simulink model "STEVE_Simulation_6DOF"  (R2025b)
settings: Solver=ode45  StartTime=0  StopTime=60  FixedStep=0.0001  MaxStep=0.0001  RelTol=1e-3
model workspace (MAT data in the model file):
  op_trim1 = opcond.OperatingReport
  op_trim1.TerminationString_ = 'Operating point specifications were successfully met.'
  op_trim1.OptimizationOutput_.iterations = 3
  op_trim1.OptimizationOutput_.funcCount = 171
  op_trim1.OptimizationOutput_.lssteplength = 1
  op_trim1.OptimizationOutput_.stepsize = 4.63262973918e-09
  op_trim1.OptimizationOutput_.algorithm = 'active-set'
  op_trim1.OptimizationOutput_.firstorderopt = 2.40097601741e-08
  op_trim1.OptimizationOutput_.constrviolation = 8.47716769092e-07
  op_trim1.OptimizationOutput_.message = 'Local minimum found that satisfies the constraints.
    | 
    | Optimization completed because the objective function is non-decreasing in 
    | feasible directions, to within the value of the optimality tolerance,
    | and constraints are satisfied to within the  value of the constraint tolerance.
    | 
    | <stopping criteria details>
    | 
    | Optimization completed: The first-order optimality measure, 2.400976e-08, is less
    | than options.OptimalityTolerance = 1.000000e-06, and the maximum constraint violation,
    | 8.477168e-07,is less than options.ConstraintTolerance = 1.000000e-06.'
  op_trim1.OptimizationOutput_.bestfeasible.x = [4290.04874097; 10725.1258376; 15852.6764872; 0.313155746169; -0.0981866680343; -0.0652604980678; 0.0059055243257; -0.636615168463; 8.14642489212e-06; -0.0176940249338; -0.00155509692213; -9.31199930506e-05; -0.000181100785288; 15.418172162; 0.559389025394; 3.31048087203; -37.2767340788; 1.38336022573; 8.21403291962e-06; 8.22046546553e-06; 8.22180678664e-06; 8.18637735168e-06; 8.165374813e-06; 8.15659926853e-06; 8.21875394544e-06; 8.19540646323e-06; 8.20244331077e-06; 8.1953609355e-06; 8.1983838895e-06; 8.22592390188e-06; 8.20694393928e-06; 8.20085018843e-06; 8.25311843786e-06; 8.2421945992e-06; 4.99999832196; 1.99999584909; 1.99999585143; 4.99999832977; 1.99999587773; 1.999995897; -0.000340053296214]
  op_trim1.OptimizationOutput_.bestfeasible.fval = 0
  op_trim1.OptimizationOutput_.bestfeasible.constrviolation = 8.47716769092e-07
  op_trim1.OptimizationOutput_.bestfeasible.firstorderopt = 2.40097601741e-08
  op_trim1.OptimizationOutput_.progress = {'<font face="monospaced"; size=3><BR>', 'Optimizing to solve for all desired dx/dt=0, x(k+1)-x(k)=0, and y=ydes.<BR>', ' <BR>', '(Maximum Error)  Block<BR>', ' ---------------------------------------------------------<BR>', '(3.86548e-01) STEVE_Simulation/STeVe System Model/Vehicle Dynamics/3DOF to 6DOF/Custom Variable Mass 3dof (Body Axes)<BR>', '(3.86551e-01) STEVE_Simulation/STeVe System Model/Vehicle Dynamics/3DOF to 6DOF/Custom Variable Mass 3dof (Body Axes)<BR>', '(8.47360e-07) STEVE_Simulation/STeVe System Model/Vehicle Dynamics/3DOF to 6DOF/Custom Variable Mass 3dof (Body Axes)<BR>', '(8.47764e-07) STEVE_Simulation/STeVe System Model/Vehicle Dynamics/3DOF to 6DOF/Custom Variable Mass 3dof (Body Axes)<BR>', '(8.47764e-07) STEVE_Simulation/STeVe System Model/Vehicle Dynamics/3DOF to 6DOF/Custom Variable Mass 3dof (Body Axes)<BR>', ' <BR>', 'Operating point specifications were successfully met.<BR>'}
  op_trim1.Model_ = 'STEVE_Simulation'
  op_trim1.States_(1) = opcond.StateReport
  op_trim1.States_(1).Nx_ = 1
  op_trim1.States_(1).Block_ = 'STEVE_Simulation/Environment/Wind/Discrete Wind Gust Model/Distance into
    | gust (x)/Distance into
    | Gust (x)
    | (Limited to gust length d)'
  op_trim1.States_(1).x_ = 1.999995897
  op_trim1.States_(1).SteadyState_ = 0
  op_trim1.States_(1).dxMin_ = -Inf
  op_trim1.States_(1).dxMax_ = Inf
  op_trim1.States_(1).Known_ = 0
  op_trim1.States_(1).Min_ = 0
  op_trim1.States_(1).Max_ = 2
  op_trim1.States_(2) = opcond.StateReport
  op_trim1.States_(2).Nx_ = 1
  op_trim1.States_(2).Block_ = 'STEVE_Simulation/Environment/Wind/Discrete Wind Gust Model/Distance into
    | gust (y)/Distance into
    | Gust (x)
    | (Limited to gust length d)
    | '
  op_trim1.States_(2).x_ = 1.99999587773
  op_trim1.States_(2).SteadyState_ = 0
  op_trim1.States_(2).dxMin_ = -Inf
  op_trim1.States_(2).dxMax_ = Inf
  op_trim1.States_(2).Known_ = 0
  op_trim1.States_(2).Min_ = 0
  op_trim1.States_(2).Max_ = 2
  op_trim1.States_(3) = opcond.StateReport
  op_trim1.States_(3).Nx_ = 1
  op_trim1.States_(3).Block_ = 'STEVE_Simulation/Environment/Wind/Discrete Wind Gust Model/Distance into
    | gust (z)/Distance into
    | Gust (x)
    | (Limited to gust length d)
    | '
  op_trim1.States_(3).x_ = 4.99999832977
  op_trim1.States_(3).SteadyState_ = 0
  op_trim1.States_(3).dxMin_ = -Inf
  op_trim1.States_(3).dxMax_ = Inf
  op_trim1.States_(3).Known_ = 0
  op_trim1.States_(3).Min_ = 0
  op_trim1.States_(3).Max_ = 5
  op_trim1.States_(4) = opcond.StateReport
  op_trim1.States_(4).Nx_ = 1
  op_trim1.States_(4).Block_ = 'STEVE_Simulation/Environment/Wind/Discrete Wind Gust Model1/Distance into
    | gust (x)/Distance into
    | Gust (x)
    | (Limited to gust length d)'
  op_trim1.States_(4).x_ = 1.99999585143
  op_trim1.States_(4).SteadyState_ = 0
  op_trim1.States_(4).dxMin_ = -Inf
  op_trim1.States_(4).dxMax_ = Inf
  op_trim1.States_(4).Known_ = 0
  op_trim1.States_(4).Min_ = 0
  op_trim1.States_(4).Max_ = 2
  op_trim1.States_(5) = opcond.StateReport
  op_trim1.States_(5).Nx_ = 1
  op_trim1.States_(5).Block_ = 'STEVE_Simulation/Environment/Wind/Discrete Wind Gust Model1/Distance into
    | gust (y)/Distance into
    | Gust (x)
    | (Limited to gust length d)
    | '
  op_trim1.States_(5).x_ = 1.99999584909
  op_trim1.States_(5).SteadyState_ = 0
  op_trim1.States_(5).dxMin_ = -Inf
  op_trim1.States_(5).dxMax_ = Inf
  op_trim1.States_(5).Known_ = 0
  op_trim1.States_(5).Min_ = 0
  op_trim1.States_(5).Max_ = 2
  op_trim1.States_(6) = opcond.StateReport
  op_trim1.States_(6).Nx_ = 1
  op_trim1.States_(6).Block_ = 'STEVE_Simulation/Environment/Wind/Discrete Wind Gust Model1/Distance into
    | gust (z)/Distance into
    | Gust (x)
    | (Limited to gust length d)
    | '
  op_trim1.States_(6).x_ = 4.99999832196
  op_trim1.States_(6).SteadyState_ = 0
  op_trim1.States_(6).dxMin_ = -Inf
  op_trim1.States_(6).dxMax_ = Inf
  op_trim1.States_(6).Known_ = 0
  op_trim1.States_(6).Min_ = 0
  op_trim1.States_(6).Max_ = 5
  op_trim1.States_(7) = opcond.StateReport
  op_trim1.States_(7).dx_ = [0; 0]
  op_trim1.States_(7).Nx_ = 2
  op_trim1.States_(7).Block_ = 'STEVE_Simulation/Environment/Wind/Dryden Wind Turbulence Model 
    | (Continuous (+q +r))/Filters on angular rates/Hpgw/pgw_p'
  op_trim1.States_(7).x_ = [8.25311843786e-06; 8.2421945992e-06]
  op_trim1.States_(7).SteadyState_ = [0; 0]
  op_trim1.States_(7).dxMin_ = [-Inf; -Inf]
  op_trim1.States_(7).dxMax_ = [Inf; Inf]
  op_trim1.States_(7).Known_ = [0; 0]
  op_trim1.States_(7).Min_ = [-Inf; -Inf]
  op_trim1.States_(7).Max_ = [Inf; Inf]
  op_trim1.States_(8) = opcond.StateReport
  op_trim1.States_(8).dx_ = [0; 0]
  op_trim1.States_(8).Nx_ = 2
  op_trim1.States_(8).Block_ = 'STEVE_Simulation/Environment/Wind/Dryden Wind Turbulence Model 
    | (Continuous (+q +r))/Filters on angular rates/Hqgw/qgw_p'
  op_trim1.States_(8).x_ = [8.20694393928e-06; 8.20085018843e-06]
  op_trim1.States_(8).SteadyState_ = [0; 0]
  op_trim1.States_(8).dxMin_ = [-Inf; -Inf]
  op_trim1.States_(8).dxMax_ = [Inf; Inf]
  op_trim1.States_(8).Known_ = [0; 0]
  op_trim1.States_(8).Min_ = [-Inf; -Inf]
  op_trim1.States_(8).Max_ = [Inf; Inf]
  op_trim1.States_(9) = opcond.StateReport
  op_trim1.States_(9).dx_ = [0; 0]
  op_trim1.States_(9).Nx_ = 2
  op_trim1.States_(9).Block_ = 'STEVE_Simulation/Environment/Wind/Dryden Wind Turbulence Model 
    | (Continuous (+q +r))/Filters on angular rates/Hrgw/rgw_p'
  op_trim1.States_(9).x_ = [8.1983838895e-06; 8.22592390188e-06]
  op_trim1.States_(9).SteadyState_ = [0; 0]
  op_trim1.States_(9).dxMin_ = [-Inf; -Inf]
  op_trim1.States_(9).dxMax_ = [Inf; Inf]
  op_trim1.States_(9).Known_ = [0; 0]
  op_trim1.States_(9).Min_ = [-Inf; -Inf]
  op_trim1.States_(9).Max_ = [Inf; Inf]
  op_trim1.States_(10) = opcond.StateReport
  op_trim1.States_(10).dx_ = [0; 0]
  op_trim1.States_(10).Nx_ = 2
  op_trim1.States_(10).Block_ = 'STEVE_Simulation/Environment/Wind/Dryden Wind Turbulence Model 
    | (Continuous (+q +r))/Filters on velocities/Hugw(s)/ug_p'
  op_trim1.States_(10).x_ = [8.20244331077e-06; 8.1953609355e-06]
  op_trim1.States_(10).SteadyState_ = [0; 0]
  op_trim1.States_(10).dxMin_ = [-Inf; -Inf]
  op_trim1.States_(10).dxMax_ = [Inf; Inf]
  op_trim1.States_(10).Known_ = [0; 0]
  op_trim1.States_(10).Min_ = [-Inf; -Inf]
  op_trim1.States_(10).Max_ = [Inf; Inf]
  op_trim1.States_(11) = opcond.StateReport
  op_trim1.States_(11).dx_ = [0; 0]
  op_trim1.States_(11).Nx_ = 2
  op_trim1.States_(11).Block_ = 'STEVE_Simulation/Environment/Wind/Dryden Wind Turbulence Model 
    | (Continuous (+q +r))/Filters on velocities/Hvgw(s)/vg_p1'
  op_trim1.States_(11).x_ = [8.165374813e-06; 8.15659926853e-06]
  op_trim1.States_(11).SteadyState_ = [0; 0]
  op_trim1.States_(11).dxMin_ = [-Inf; -Inf]
  op_trim1.States_(11).dxMax_ = [Inf; Inf]
  op_trim1.States_(11).Known_ = [0; 0]
  op_trim1.States_(11).Min_ = [-Inf; -Inf]
  op_trim1.States_(11).Max_ = [Inf; Inf]
  op_trim1.States_(12) = opcond.StateReport
  op_trim1.States_(12).dx_ = [0; 0]
  op_trim1.States_(12).Nx_ = 2
  op_trim1.States_(12).Block_ = 'STEVE_Simulation/Environment/Wind/Dryden Wind Turbulence Model 
    | (Continuous (+q +r))/Filters on velocities/Hvgw(s)/vgw_p2'
  op_trim1.States_(12).x_ = [8.21875394544e-06; 8.19540646323e-06]
  op_trim1.States_(12).SteadyState_ = [0; 0]
  op_trim1.States_(12).dxMin_ = [-Inf; -Inf]
  op_trim1.States_(12).dxMax_ = [Inf; Inf]
  op_trim1.States_(12).Known_ = [0; 0]
  op_trim1.States_(12).Min_ = [-Inf; -Inf]
  op_trim1.States_(12).Max_ = [Inf; Inf]
  op_trim1.States_(13) = opcond.StateReport
  op_trim1.States_(13).dx_ = [0; 0]
  op_trim1.States_(13).Nx_ = 2
  op_trim1.States_(13).Block_ = 'STEVE_Simulation/Environment/Wind/Dryden Wind Turbulence Model 
    | (Continuous (+q +r))/Filters on velocities/Hwgw(s)/wg_p1'
  op_trim1.States_(13).x_ = [8.21403291962e-06; 8.22046546553e-06]
  op_trim1.States_(13).SteadyState_ = [0; 0]
  op_trim1.States_(13).dxMin_ = [-Inf; -Inf]
  op_trim1.States_(13).dxMax_ = [Inf; Inf]
  op_trim1.States_(13).Known_ = [0; 0]
  op_trim1.States_(13).Min_ = [-Inf; -Inf]
  op_trim1.States_(13).Max_ = [Inf; Inf]
  op_trim1.States_(14) = opcond.StateReport
  op_trim1.States_(14).dx_ = [0; 0]
  op_trim1.States_(14).Nx_ = 2
  op_trim1.States_(14).Block_ = 'STEVE_Simulation/Environment/Wind/Dryden Wind Turbulence Model 
    | (Continuous (+q +r))/Filters on velocities/Hwgw(s)/wg_p2'
  op_trim1.States_(14).x_ = [8.22180678664e-06; 8.18637735168e-06]
  op_trim1.States_(14).SteadyState_ = [0; 0]
  op_trim1.States_(14).dxMin_ = [-Inf; -Inf]
  op_trim1.States_(14).dxMax_ = [Inf; Inf]
  op_trim1.States_(14).Known_ = [0; 0]
  op_trim1.States_(14).Min_ = [-Inf; -Inf]
  op_trim1.States_(14).Max_ = [Inf; Inf]
  op_trim1.States_(15) = opcond.StateReport
  op_trim1.States_(15).dx_ = [-1624.62107391; 4290.04874097; 10725.1258376]
  op_trim1.States_(15).Nx_ = 3
  op_trim1.States_(15).Block_ = 'STEVE_Simulation/GuidanceCommands/Transfer Fcn'
  op_trim1.States_(15).x_ = [4290.04874097; 10725.1258376; 15852.6764872]
  op_trim1.States_(15).SteadyState_ = [0; 0; 0]
  op_trim1.States_(15).dxMin_ = [-Inf; -Inf; -Inf]
  op_trim1.States_(15).dxMax_ = [Inf; Inf; Inf]
  op_trim1.States_(15).Known_ = [0; 0; 0]
  op_trim1.States_(15).Min_ = [-Inf; -Inf; -Inf]
  op_trim1.States_(15).Max_ = [Inf; Inf; Inf]
  op_trim1.States_(16) = opcond.StateReport
  op_trim1.States_(16).dx_ = -3.37116243602
  op_trim1.States_(16).Nx_ = 1
  op_trim1.States_(16).Block_ = 'STEVE_Simulation/STeVe System Model/Control System/Classical Upgraded/PID Controller1/Filter/Cont. Filter/Filter'
  op_trim1.States_(16).x_ = -0.00155509692213
  op_trim1.States_(16).SteadyState_ = 0
  op_trim1.States_(16).dxMin_ = -Inf
  op_trim1.States_(16).dxMax_ = Inf
  op_trim1.States_(16).Known_ = 0
  op_trim1.States_(16).Min_ = -Inf
  op_trim1.States_(16).Max_ = Inf
  op_trim1.States_(17) = opcond.StateReport
  op_trim1.States_(17).dx_ = -0.00991390700733
  op_trim1.States_(17).Nx_ = 1
  op_trim1.States_(17).Block_ = 'STEVE_Simulation/STeVe System Model/Control System/Classical Upgraded/PID Controller1/Integrator/Continuous/Integrator'
  op_trim1.States_(17).x_ = -0.0176940249338
  op_trim1.States_(17).SteadyState_ = 0
  op_trim1.States_(17).dxMin_ = -Inf
  op_trim1.States_(17).dxMax_ = Inf
  op_trim1.States_(17).Known_ = 0
  op_trim1.States_(17).Min_ = -Inf
  op_trim1.States_(17).Max_ = Inf
  op_trim1.States_(18) = opcond.StateReport
  op_trim1.States_(18).dx_ = 0.00151513100245
  op_trim1.States_(18).Nx_ = 1
  op_trim1.States_(18).Block_ = 'STEVE_Simulation/STeVe System Model/Control System/Classical Upgraded/PID Controller2/Filter/Cont. Filter/Filter'
  op_trim1.States_(18).x_ = 0.0059055243257
  op_trim1.States_(18).SteadyState_ = 0
  op_trim1.States_(18).dxMin_ = -Inf
  op_trim1.States_(18).dxMax_ = Inf
  op_trim1.States_(18).Known_ = 0
  op_trim1.States_(18).Min_ = -Inf
  op_trim1.States_(18).Max_ = Inf
  op_trim1.States_(19) = opcond.StateReport
  op_trim1.States_(19).dx_ = -0.037481221471
  op_trim1.States_(19).Nx_ = 1
  op_trim1.States_(19).Block_ = 'STEVE_Simulation/STeVe System Model/Control System/Classical Upgraded/PID Controller2/Integrator/Continuous/Integrator'
  op_trim1.States_(19).x_ = -0.0652604980678
  op_trim1.States_(19).SteadyState_ = 0
  op_trim1.States_(19).dxMin_ = -Inf
  op_trim1.States_(19).dxMax_ = Inf
  op_trim1.States_(19).Known_ = 0
  op_trim1.States_(19).Min_ = -Inf
  op_trim1.States_(19).Max_ = Inf
  op_trim1.States_(20) = opcond.StateReport
  op_trim1.States_(20).dx_ = -0.0747869203805
  op_trim1.States_(20).Nx_ = 1
  op_trim1.States_(20).Block_ = 'STEVE_Simulation/STeVe System Model/Control System/Classical Upgraded/PID Controller3/Filter/Cont. Filter/Filter'
  op_trim1.States_(20).x_ = -0.0981866680343
  op_trim1.States_(20).SteadyState_ = 0
  op_trim1.States_(20).dxMin_ = -Inf
  op_trim1.States_(20).dxMax_ = Inf
  op_trim1.States_(20).Known_ = 0
  op_trim1.States_(20).Min_ = -Inf
  op_trim1.States_(20).Max_ = Inf
  op_trim1.States_(21) = opcond.StateReport
  op_trim1.States_(21).dx_ = 0.273198142244
  op_trim1.States_(21).Nx_ = 1
  op_trim1.States_(21).Block_ = 'STEVE_Simulation/STeVe System Model/Control System/Classical Upgraded/PID Controller3/Integrator/Continuous/Integrator'
  op_trim1.States_(21).x_ = 0.313155746169
  op_trim1.States_(21).SteadyState_ = 0
  op_trim1.States_(21).dxMin_ = -Inf
  op_trim1.States_(21).dxMax_ = Inf
  op_trim1.States_(21).Known_ = 0
  op_trim1.States_(21).Min_ = -Inf
  op_trim1.States_(21).Max_ = Inf
  op_trim1.States_(22) = opcond.StateReport
  op_trim1.States_(22).dx_ = -0.000814642489212
  op_trim1.States_(22).Nx_ = 1
  op_trim1.States_(22).Block_ = 'STEVE_Simulation/STeVe System Model/Control System/Classical Upgraded/PID Controller6/Filter/Cont. Filter/Filter'
  op_trim1.States_(22).x_ = 8.14642489212e-06
  op_trim1.States_(22).SteadyState_ = 0
  op_trim1.States_(22).dxMin_ = -Inf
  op_trim1.States_(22).dxMax_ = Inf
  op_trim1.States_(22).Known_ = 0
  op_trim1.States_(22).Min_ = -Inf
  op_trim1.States_(22).Max_ = Inf
  op_trim1.States_(23) = opcond.StateReport
  op_trim1.States_(23).dx_ = -0.133481022202
  op_trim1.States_(23).Nx_ = 1
  op_trim1.States_(23).Block_ = 'STEVE_Simulation/STeVe System Model/Control System/Classical Upgraded/PID Controller6/Integrator/Continuous/Integrator'
  op_trim1.States_(23).x_ = -0.636615168463
  op_trim1.States_(23).SteadyState_ = 0
  op_trim1.States_(23).dxMin_ = -Inf
  op_trim1.States_(23).dxMax_ = Inf
  op_trim1.States_(23).Known_ = 0
  op_trim1.States_(23).Min_ = -Inf
  op_trim1.States_(23).Max_ = Inf
  op_trim1.States_(24) = opcond.StateReport
  op_trim1.States_(24).dx_ = 3.05199662227
  op_trim1.States_(24).Nx_ = 1
  op_trim1.States_(24).Block_ = 'STEVE_Simulation/STeVe System Model/Vehicle Dynamics/3DOF to 6DOF/Custom Variable Mass 3dof
    | (Body Axes)'
  op_trim1.States_(24).StateName_ = 'u'
  op_trim1.States_(24).x_ = 15.418172162
  op_trim1.States_(24).SteadyState_ = 0
  op_trim1.States_(24).dxMin_ = -Inf
  op_trim1.States_(24).dxMax_ = Inf
  op_trim1.States_(24).Known_ = 0
  op_trim1.States_(24).Min_ = -Inf
  op_trim1.States_(24).Max_ = Inf
  op_trim1.States_(25) = opcond.StateReport
  op_trim1.States_(25).dx_ = 1.82984252685
  op_trim1.States_(25).Nx_ = 1
  op_trim1.States_(25).Block_ = 'STEVE_Simulation/STeVe System Model/Vehicle Dynamics/3DOF to 6DOF/Custom Variable Mass 3dof
    | (Body Axes)'
  op_trim1.States_(25).StateName_ = 'w'
  op_trim1.States_(25).x_ = 0.559389025394
  op_trim1.States_(25).SteadyState_ = 0
  op_trim1.States_(25).dxMin_ = -Inf
  op_trim1.States_(25).dxMax_ = Inf
  op_trim1.States_(25).Known_ = 0
  op_trim1.States_(25).Min_ = -Inf
  op_trim1.States_(25).Max_ = Inf
  op_trim1.States_(26) = opcond.StateReport
  op_trim1.States_(26).dx_ = 3.42262162857
  op_trim1.States_(26).Nx_ = 1
  op_trim1.States_(26).Block_ = 'STEVE_Simulation/STeVe System Model/Vehicle Dynamics/3DOF to 6DOF/Custom Variable Mass 3dof
    | (Body Axes)'
  op_trim1.States_(26).StateName_ = 'Xe'
  op_trim1.States_(26).x_ = 3.31048087203
  op_trim1.States_(26).SteadyState_ = 0
  op_trim1.States_(26).dxMin_ = -Inf
  op_trim1.States_(26).dxMax_ = Inf
  op_trim1.States_(26).Known_ = 0
  op_trim1.States_(26).Min_ = -Inf
  op_trim1.States_(26).Max_ = Inf
  op_trim1.States_(27) = opcond.StateReport
  op_trim1.States_(27).dx_ = -15.0438894601
  op_trim1.States_(27).Nx_ = 1
  op_trim1.States_(27).Block_ = 'STEVE_Simulation/STeVe System Model/Vehicle Dynamics/3DOF to 6DOF/Custom Variable Mass 3dof
    | (Body Axes)'
  op_trim1.States_(27).StateName_ = 'Ze'
  op_trim1.States_(27).x_ = -37.2767340788
  op_trim1.States_(27).SteadyState_ = 0
  op_trim1.States_(27).dxMin_ = -Inf
  op_trim1.States_(27).dxMax_ = Inf
  op_trim1.States_(27).Known_ = 0
  op_trim1.States_(27).Min_ = -Inf
  op_trim1.States_(27).Max_ = Inf
  op_trim1.States_(28) = opcond.StateReport
  op_trim1.States_(28).dx_ = 8.47764429975e-07
  op_trim1.States_(28).Nx_ = 1
  op_trim1.States_(28).Block_ = 'STEVE_Simulation/STeVe System Model/Vehicle Dynamics/3DOF to 6DOF/Custom Variable Mass 3dof
    | (Body Axes)'
  op_trim1.States_(28).StateName_ = 'q'
  op_trim1.States_(28).SteadyState_ = 1
  op_trim1.States_(28).dxMin_ = -Inf
  op_trim1.States_(28).dxMax_ = Inf
  op_trim1.States_(28).Known_ = 1
  op_trim1.States_(28).Min_ = -Inf
  op_trim1.States_(28).Max_ = Inf
  op_trim1.States_(29) = opcond.StateReport
  op_trim1.States_(29).Nx_ = 1
  op_trim1.States_(29).Block_ = 'STEVE_Simulation/STeVe System Model/Vehicle Dynamics/3DOF to 6DOF/Custom Variable Mass 3dof
    | (Body Axes)'
  op_trim1.States_(29).StateName_ = 'theta'
  op_trim1.States_(29).x_ = 1.38336022573
  op_trim1.States_(29).SteadyState_ = 1
  op_trim1.States_(29).dxMin_ = -Inf
  op_trim1.States_(29).dxMax_ = Inf
  op_trim1.States_(29).Known_ = 0
  op_trim1.States_(29).Min_ = -Inf
  op_trim1.States_(29).Max_ = Inf
  op_trim1.States_(30) = opcond.StateReport
  op_trim1.States_(30).dx_ = -3.39724258746
  op_trim1.States_(30).Nx_ = 1
  op_trim1.States_(30).Block_ = 'STEVE_Simulation/STeVe System Model/Vehicle Dynamics/RocketEngineActuators/Delay'
  op_trim1.States_(30).x_ = -0.000340053296214
  op_trim1.States_(30).Ts_ = [0.0001 0]
  op_trim1.States_(30).SampleType_ = 'DSTATE'
  op_trim1.States_(30).SteadyState_ = 0
  op_trim1.States_(30).dxMin_ = -Inf
  op_trim1.States_(30).dxMax_ = Inf
  op_trim1.States_(30).Known_ = 0
  op_trim1.States_(30).Min_ = -Inf
  op_trim1.States_(30).Max_ = Inf
  op_trim1.States_(31) = opcond.StateReport
  op_trim1.States_(31).dx_ = [-0.000181100785288; -0.936056601197]
  op_trim1.States_(31).Nx_ = 2
  op_trim1.States_(31).Block_ = 'STEVE_Simulation/STeVe System Model/Vehicle Dynamics/RocketEngineActuators/Servo/Integrator,
    | Second-Order
    | Limited'
  op_trim1.States_(31).x_ = [-9.31199930506e-05; -0.000181100785288]
  op_trim1.States_(31).SteadyState_ = [0; 0]
  op_trim1.States_(31).dxMin_ = [-Inf; -Inf]
  op_trim1.States_(31).dxMax_ = [Inf; Inf]
  op_trim1.States_(31).Known_ = [0; 0]
  op_trim1.States_(31).Min_ = [-Inf; -Inf]
  op_trim1.States_(31).Max_ = [Inf; Inf]
undefined symbols (not defined in the file): Actuators, AeroData, C_inner_maxQ_d_Ki, C_inner_maxQ_d_Kp, C_outer_maxQ_d_Ki, C_outer_maxQ_d_Kp, F, launchpad_alt, Light, MIL, PrelookupData, Ref_Area, rocket_length, timeStep, Ts_inner, Ts_outer, warm_up_time, wn_ramp
libraries: simulink_extras x23, simulink x7, slpidlib x5, aerolibwind2 x3, aerolibconvert2 x3, aerolibasang x2, aerolibactuator x2, aerolibatmos2 x1
(part 1 of 2)
settings Model: SimulationMode=accelerator  ExtModeTrigDuration=2  Creator=jonno  LastModifiedBy=jonno
settings SolverCC: AutoInsertRateTranBlk=on
settings DataIOCC: ExternalInput=getinputstruct(op_trim1)  InitialState=getstatestruct(op_trim1)  SaveFormat=StructureWithTime
settings OptimizationCC: BlockReduction=off  BufferReuse=off
settings DebuggingCC: AlgebraicLoopMsg=none
settings HardwareCC: ProdBitPerLong=64.0  ProdHWDeviceType=Apple->ARM64
settings RTWCC: BuildConfiguration=Faster Runs
settings GRTTargetCC: RTWCAPISignals=on  RTWCAPIParams=on
settings ExplorerConfigSet: SimMechanicsOpenEditorOnUpdate=off

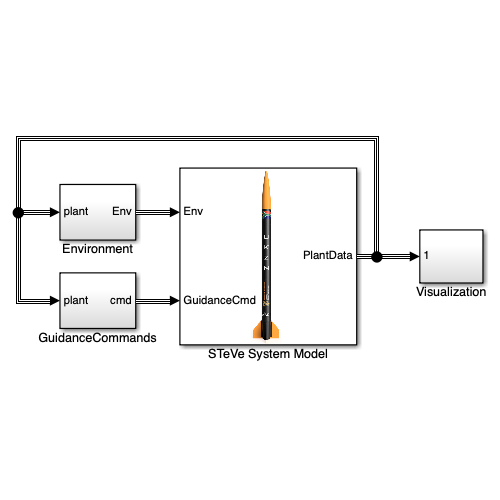
[thumbnail: Simulink's stored preview of the top-level diagram]
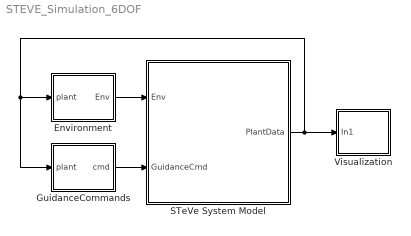
== system STEVE_Simulation_6DOF ==
  Environment : Subsystem
  GuidanceCommands : Subsystem
  STeVe System Model : Subsystem
      mask Display: image('/Users/jonno/MATLAB-Drive/masters-rocket-control-repository/simulation_6dof/docs/images/steve.png', [65 - (50 * (187 / 1041)), 0, 140 * (187 / 1041), 140])
  Visualization : Subsystem
  wires:
  GuidanceCommands/1(cmd) -> STeVe System Model/2(GuidanceCmd)
  Environment/1(Env) -> STeVe System Model/1(Env)
  STeVe System Model/1(PlantData) -> GuidanceCommands/1(plant), Environment/1(plant), Visualization/1(In1)

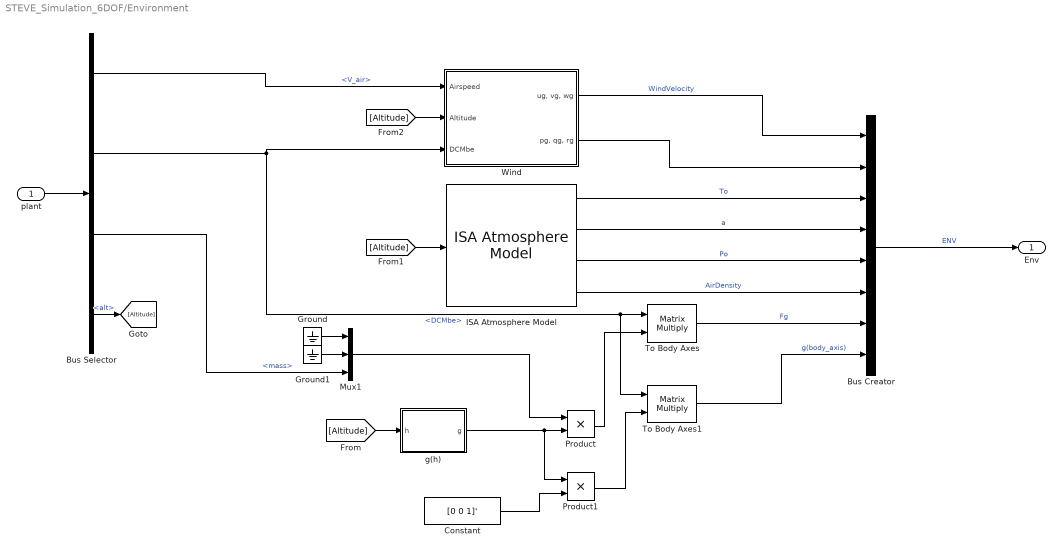
== system STEVE_Simulation_6DOF/Environment ==
  plant : Inport
  Bus Creator : BusCreator  Inputs=8
  Bus Selector : BusSelector  OutputSignals=V_air,DCMbe,mass,alt
  Constant : Constant  Value=[0 0 1]'
  Ground : Ground
  Ground1 : Ground
  ISA Atmosphere Model : aerolibatmos2/ISA Atmosphere Model  useExtended=on  action=None  custom=off  viscosityOut=off  g=9.80665  gamma=1.4  R=287.0531  L=0.0065  h_trop=11000  h_strat=20000  rho0=1.225  P0=101325  T0=288.15  h0=0  S=110.4  Tref=273.15  muref=1.716e-5
  Mux1 : Mux  Inputs=3
  Product : Product
  Product1 : Product
  To Body Axes : Product  Multiplication=Matrix(*)
  To Body Axes1 : Product  Multiplication=Matrix(*)
  Wind : Subsystem
  g(h) : MATLAB Function  TreatAsAtomicUnit=on
  Env : Outport
  wires:
  plant/1 -> Bus Selector/1
  Bus Creator/1 -> Env/1  "ENV"
  Bus Selector/3 -> Mux1/3  "<mass>"
  Ground/1 -> Mux1/1
  Ground1/1 -> Mux1/2
  Bus Selector/2 -> Wind/3(DCMbe), To Body Axes1/1, To Body Axes/1  "<DCMbe>"
  [Altitude] -> ISA Atmosphere Model/1
  To Body Axes/1 -> Bus Creator/7  "Fg"
  ISA Atmosphere Model/4 -> Bus Creator/6  "AirDensity"
  ISA Atmosphere Model/3 -> Bus Creator/5  "Po"
  ISA Atmosphere Model/2 -> Bus Creator/4  "a"
  ISA Atmosphere Model/1 -> Bus Creator/3  "To"
  [Altitude] -> Wind/2(Altitude)
  Wind/2("pg, qg, rg") -> Bus Creator/2
  Mux1/1 -> Product/1
  Product/1 -> To Body Axes/2
  [Altitude] -> g(h)/1(h)
  g(h)/1(g) -> Product1/1, Product/2
  Wind/1("ug, vg, wg") -> Bus Creator/1  "WindVelocity"
  Constant/1 -> Product1/2
  Product1/1 -> To Body Axes1/2
  To Body Axes1/1 -> Bus Creator/8  "g(body_axis)"
  Bus Selector/4 -> [Altitude]  "<alt>"
  Bus Selector/1 -> Wind/1(Airspeed)  "<V_air>"

== system STEVE_Simulation_6DOF/GuidanceCommands ==
  plant : Inport
  Bus Creator : BusCreator  Inputs=4
  Constant : Constant  Value=90
  Constant1 : Constant  Value=0
  Degrees to Radians : simulink_extras/Transformations/Degrees to Radians
  Degrees to Radians1 : simulink_extras/Transformations/Degrees to Radians
  Rate Limiter : RateLimiter  RisingSlewLimit=2000/60  FallingSlewLimit=-0.5  SampleTimeMode=inherited
  Rate Limiter2 : RateLimiter  RisingSlewLimit=0.5  FallingSlewLimit=-0.5  SampleTimeMode=inherited
  Step : Step  After=2000  SampleTime=0
  ThrottleCmd % : Step  Time=Actuators.Engine.BurnTime  Before=1  After=0.0001  SampleTime=0  VectorParams1D=off
  cmd : Outport
  wires:
  Bus Creator/1 -> cmd/1  "CMD"
  Degrees to Radians/1 -> Bus Creator/2  "theta_cmd"
  ThrottleCmd %/1 -> Rate Limiter2/1  "ThrottleCmd"
  Rate Limiter2/1 -> Bus Creator/1  "throttle_cmd"
  Constant/1 -> Degrees to Radians/1
  Step/1 -> Rate Limiter/1
  Rate Limiter/1 -> Bus Creator/4  "Xe_Cmd"
  Constant1/1 -> Degrees to Radians1/1
  Degrees to Radians1/1 -> Bus Creator/3  "psi_cmd"

== system STEVE_Simulation_6DOF/STeVe System Model ==
  Env : Inport
  GuidanceCmd : Inport  Port=2
  Env1 : InportShadow
  State Estimator : Subsystem
  Subsystem : Subsystem
  Vehicle Dynamics : Subsystem
  PlantData : Outport
  wires:
  Env/1 -> Vehicle Dynamics/1(Env)
  Vehicle Dynamics/1(PlantData) -> Subsystem/3(PlantData), State Estimator/2(Plant), PlantData/1  "Plant"
  GuidanceCmd/1 -> Subsystem/1(GuidanceCommandBus)
  Env1/1 -> State Estimator/1(Env)
  State Estimator/1(Sensors) -> Subsystem/2(Sensors)
  Subsystem/1(ActCmd) -> Vehicle Dynamics/2(ActCmd)

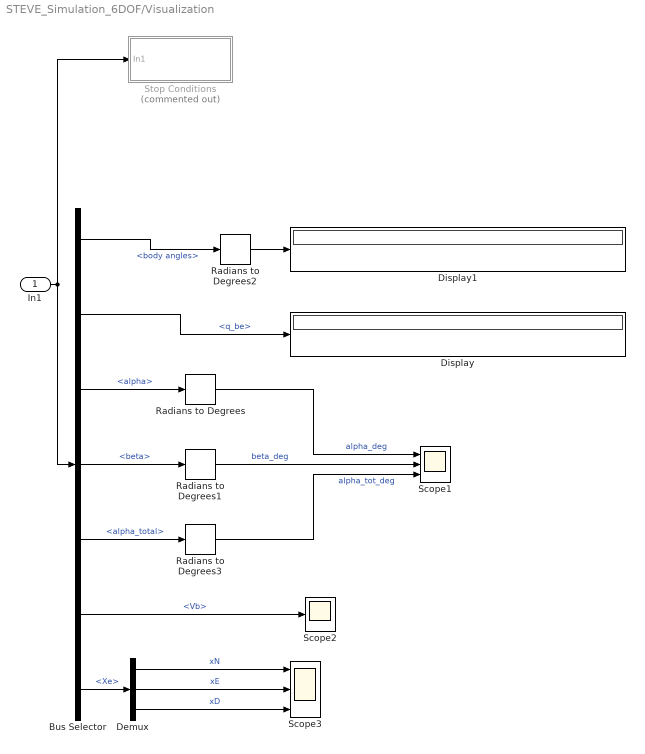
== system STEVE_Simulation_6DOF/Visualization ==
  In1 : Inport
  Bus Selector : BusSelector  OutputSignals=body angles,q_be,alpha,beta,alpha_total,Vb,Xe
  Demux : Demux  Outputs=3
  Display : Display
  Display1 : Display
  Radians to Degrees{,1..3} (4 alike) : simulink_extras/Transformations/Radians to Degrees
  Scope1 : Scope  NumInputPorts=3
      settings: ActiveDisplayYMinimum=0.52794946772114626  ActiveDisplayYMaximum=0.85095852928901983  DataLoggingVariableName=ScopeData3
  Scope2 : Scope
      settings: ActiveDisplayYMinimum=-0.64239324283240506  ActiveDisplayYMaximum=0.59138262660134089  DataLoggingVariableName=ScopeData4
  Scope3 : Scope  NumInputPorts=3
      settings: ActiveDisplayYMinimum=-1.7095998760294862  ActiveDisplayYMaximum=2.8596467575037732
  Stop Conditions : Subsystem  Commented=on
  wires:
  In1/1 -> Stop Conditions/1(In1), Bus Selector/1
  Bus Selector/1 -> Radians to Degrees2/1  "<body angles>"
  Bus Selector/3 -> Radians to Degrees/1  "<alpha>"
  Bus Selector/4 -> Radians to Degrees1/1  "<beta>"
  Radians to Degrees/1 -> Scope1/1  "alpha_deg"
  Radians to Degrees1/1 -> Scope1/2  "beta_deg"
  Bus Selector/6 -> Scope2/1  "<Vb>"
  Bus Selector/2 -> Display/1  "<q_be>"
  Radians to Degrees2/1 -> Display1/1
  Bus Selector/7 -> Demux/1  "<Xe>"
  Demux/2 -> Scope3/2  "xE"
  Demux/1 -> Scope3/1  "xN"
  Demux/3 -> Scope3/3  "xD"
  Bus Selector/5 -> Radians to Degrees3/1  "<alpha_total>"
  Radians to Degrees3/1 -> Scope1/3  "alpha_tot_deg"

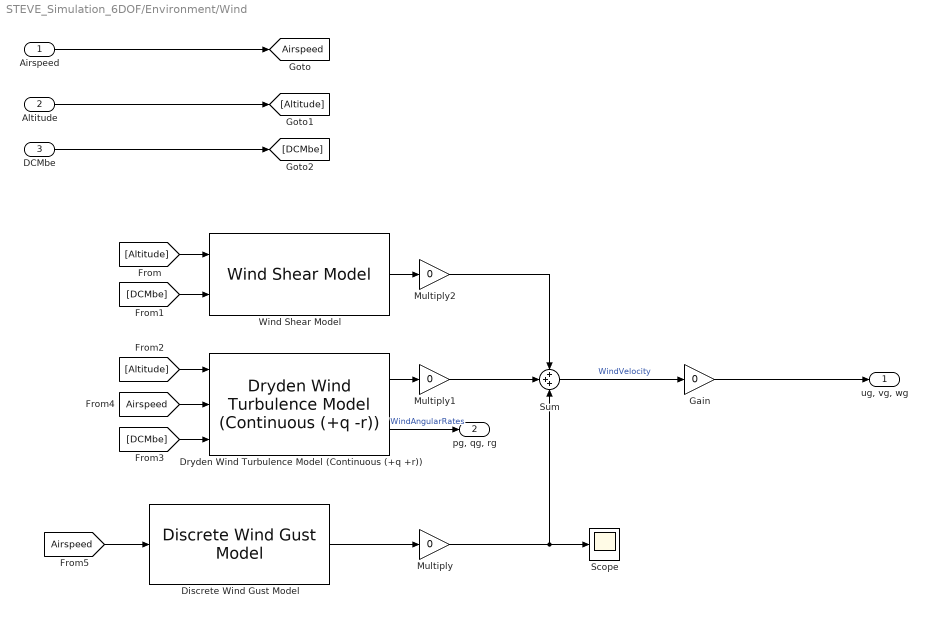
== system STEVE_Simulation_6DOF/Environment/Wind ==
  Airspeed : Inport
  Altitude : Inport  Port=2
  DCMbe : Inport  Port=3
  Discrete Wind Gust Model : aerolibwind2/Discrete Wind Gust Model  units=Metric (MKS)  Gx=on  Gy=off  Gz=off  t_0=1  d_m=[50 10 10]  v_m=[30 0 0]
  Dryden Wind Turbulence Model (Continuous (+q +r)) : aerolibwind2/Dryden Wind Turbulence Model  (Continuous (+q -r))  units=Metric (MKS)  spec=MIL-F-8785C  model=Continuous Dryden (+q +r)  W20=15  Wdeg=0  TurbProb=10^-2 - Light  L_high=533.4  Wingspan=10  ts=0.1  Seed=[23341 23342 23343 23344]  T_on=off
      settings: LibrarySourceBlock=|
      | aerolibwind2/Dryden Wind Turbulence Model
      | (Continuous (+q +r))
  Gain : Gain  Gain=0
  Multiply : Gain  Gain=0
  Multiply1 : Gain  Gain=0
  Multiply2 : Gain  Gain=0
  Scope : Scope
      settings: ActiveDisplayYMinimum=-3.4473346269998206  ActiveDisplayYMaximum=16.02681366587808  DataLoggingVariableName=ScopeData5
  Sum : Sum  Inputs=+++
  Wind Shear Model : aerolibwind2/Wind Shear Model  units=Metric (MKS)  phase=Category C - Terminal Flight Phase  W_20=Wind.shear  Wdeg=90
  "ug, vg, wg" : Outport
  "pg, qg, rg" : Outport  Port=2
  tag scope: Airspeed=global
  wires:
  DCMbe/1 -> [DCMbe]
  [Altitude] -> Wind Shear Model/1
  [DCMbe] -> Wind Shear Model/2
  [Altitude] -> Dryden Wind Turbulence Model (Continuous (+q +r))/1
  [DCMbe] -> Dryden Wind Turbulence Model (Continuous (+q +r))/3
  [Airspeed] -> Dryden Wind Turbulence Model (Continuous (+q +r))/2
  [Airspeed] -> Discrete Wind Gust Model/1
  Sum/1 -> Gain/1  "WindVelocity"
  Dryden Wind Turbulence Model (Continuous (+q +r))/2 -> "pg, qg, rg"/1  "WindAngularRates"
  Altitude/1 -> [Altitude]
  Multiply/1 -> Sum/3, Scope/1
  Wind Shear Model/1 -> Multiply2/1
  Dryden Wind Turbulence Model (Continuous (+q +r))/1 -> Multiply1/1
  Multiply1/1 -> Sum/2
  Multiply2/1 -> Sum/1
  Discrete Wind Gust Model/1 -> Multiply/1
  Airspeed/1 -> [Airspeed]
  Gain/1 -> "ug, vg, wg"/1

== system STEVE_Simulation_6DOF/STeVe System Model/State Estimator ==
  note: We need to estimate Qbar
  Env : Inport
  Plant : Inport  Port=2
  Bus Creator : BusCreator  Inputs=3
  Bus Selector : BusSelector  OutputSignals=lat,long,alt,Ve,Ab,w,DCMbe,body angles,V_air
  Bus Selector1 : BusSelector  OutputSignals=g(body_axis),AirDensity
  Sensors : Outport
  wires:
  Plant/1 -> Bus Selector/1
  Env/1 -> Bus Selector1/1
  Bus Creator/1 -> Sensors/1
  [qbar] -> Bus Creator/3

== system STEVE_Simulation_6DOF/STeVe System Model/Subsystem ==
  GuidanceCommandBus : Inport
  Sensors : Inport  Port=2
  PlantData : Inport  Port=3
  Classical Upgraded : Subsystem
  Classical Upgraded1 : Subsystem  Commented=on
  ActCmd : Outport
  wires:
  Sensors/1 -> Classical Upgraded/2(Sensors)
  PlantData/1 -> Classical Upgraded/1(PlantData)
  Classical Upgraded/1(Cmd Out) -> ActCmd/1
  GuidanceCommandBus/1 -> Classical Upgraded/3(CMD)

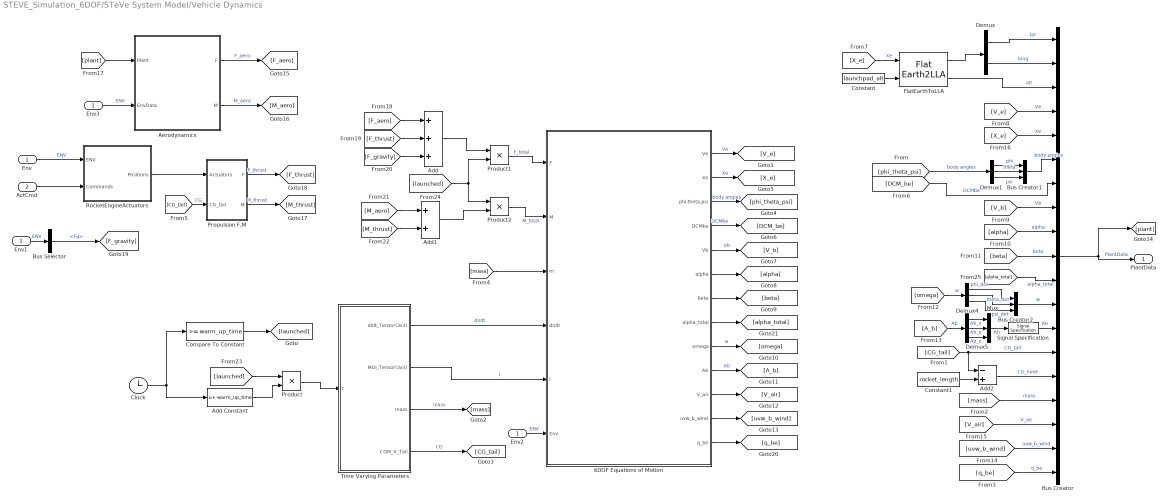
== system STEVE_Simulation_6DOF/STeVe System Model/Vehicle Dynamics ==
  Env : Inport
  ActCmd : Inport  Port=2
  6DOF Equations of Motion : Subsystem
  Add : Sum  Inputs=+++
  Add Constant : Bias  Bias=-warm_up_time  SaturateOnIntegerOverflow=off
  Add1 : Sum
  Add2 : Sum  Inputs=-+
  Aerodynamics : Subsystem
  Bus Creator : BusCreator  Inputs=19
  Bus Creator1 : BusCreator  Inputs=3
  Bus Creator2 : BusCreator  Inputs=3
  Bus Selector : BusSelector  OutputSignals=Fg
  Clock : Clock
  Compare To Constant : simulink/Logic and Bit Operations/Compare To Constant  relop=>=  const=warm_up_time  OutDataTypeStr=boolean
  Constant : Constant  Value=launchpad_alt
  Constant1 : Constant  Value=rocket_length
  Demux : Demux  Outputs=2
  Demux1 : Demux  Outputs=3
  Demux4 : Demux  Outputs=3
  Demux5 : Demux  Outputs=3
  Env1 : InportShadow
  Env2 : InportShadow
  Env3 : InportShadow
  FlatEarthToLLA : FlatEarth2LLA  R=6378137
  Mux : Mux  Inputs=3
  Product : Product
  Product1 : Product
  Product2 : Product
  Propulsion F,M : Subsystem
  RocketEngineActuators : Subsystem
  Signal Specification : SignalSpecification  Dimensions=[1 3]
  Time Varying Parameters : Subsystem
  PlantData : Outport
  wires:
  ActCmd/1 -> RocketEngineActuators/2(Commands)
  RocketEngineActuators/1(Positions) -> Propulsion F,M/1(Actuators)
  Bus Creator/1 -> [plant], PlantData/1  "PlantData"
  [X_e] -> FlatEarthToLLA/1  "Xe"
  Demux/1 -> Bus Creator/1  "lat"
  Demux/2 -> Bus Creator/2  "long"
  FlatEarthToLLA/1 -> Demux/1
  FlatEarthToLLA/2 -> Bus Creator/3  "alt"
  [V_e] -> Bus Creator/4  "Ve"
  [phi_theta_psi] -> Demux1/1  "body angles"
  Demux1/1 -> Bus Creator1/1  "phi"
  Demux1/2 -> Bus Creator1/2  "theta"
  Demux1/3 -> Bus Creator1/3  "psi"
  Bus Creator1/1 -> Bus Creator/6  "body angles"
  [DCM_be] -> Bus Creator/7  "DCMbe"
  [V_b] -> Bus Creator/8  "Vb"
  [alpha] -> Bus Creator/9  "alpha"
  [beta] -> Bus Creator/10  "beta"
  [omega] -> Demux4/1  "w"
  Signal Specification/1 -> Bus Creator/13  "Ab"
  Propulsion F,M/1(F) -> [F_thrust]  "F_thrust"
  [CG_tail] -> Bus Creator/14, Add2/1  "CG_tail"
  [mass] -> Bus Creator/16  "mass"
  Env/1 -> RocketEngineActuators/1(ENV)  "ENV"
  Propulsion F,M/2(M) -> [M_thrust]  "M_thrust"
  Clock/1 -> Add Constant/1, Compare To Constant/1
  Time Varying Parameters/1(dIdt_Tensor(3x3)) -> 6DOF Equations of Motion/4(dI/dt)  "dI/dt"
  Time Varying Parameters/2(MOI_Tensor(3x3)) -> 6DOF Equations of Motion/5(I)  "I"
  Time Varying Parameters/3(mass) -> [mass]  "mass"
  Time Varying Parameters/4(COM_X_Tail) -> [CG_tail]  "CG"
  [mass] -> 6DOF Equations of Motion/3(m)
  Product1/1 -> 6DOF Equations of Motion/1(F)  "F_total"
  Aerodynamics/1(F) -> [F_aero]  "F_aero"
  Env2/1 -> 6DOF Equations of Motion/6(Env)  "ENV"
  [CG_tail] -> Propulsion F,M/2(CG_tail)  "CG"
  Aerodynamics/2(M) -> [M_aero]  "M_aero"
  [uvw_b_wind] -> Bus Creator/18  "uvw_b_wind"
  Demux4/1 -> Bus Creator2/1  "phi_dot"
  Demux4/3 -> Bus Creator2/3  "psi_dot"
  Demux4/2 -> Bus Creator2/2  "theta_dot"
  Bus Creator2/1 -> Bus Creator/12  "w"
  Demux5/1 -> Mux/1  "Ab_x"
  Demux5/2 -> Mux/2  "Ab_y"
  Demux5/3 -> Mux/3  "Ab_z"
  [A_b] -> Demux5/1  "Ab"
  Mux/1 -> Signal Specification/1  "Ab"
  Product2/1 -> 6DOF Equations of Motion/2(M)  "M_total"
  Constant/1 -> FlatEarthToLLA/2
  6DOF Equations of Motion/1(Ve) -> [V_e]  "Ve"
  6DOF Equations of Motion/3(phi,theta,psi) -> [phi_theta_psi]  "body angles"
  6DOF Equations of Motion/2(Xe) -> [X_e]  "Xe"
  6DOF Equations of Motion/4(DCMbe) -> [DCM_be]  "DCMbe"
  6DOF Equations of Motion/5(Vb) -> [V_b]  "Vb"
  6DOF Equations of Motion/6(alpha) -> [alpha]
  6DOF Equations of Motion/7(beta) -> [beta]
  6DOF Equations of Motion/9(omega) -> [omega]  "w"
  6DOF Equations of Motion/10(Ab) -> [A_b]  "Ab"
  6DOF Equations of Motion/11(V_air) -> [V_air]
  6DOF Equations of Motion/12(uvw_b_wind) -> [uvw_b_wind]
  [V_air] -> Bus Creator/17  "V_air"
  [X_e] -> Bus Creator/5  "Xe"
  [plant] -> Aerodynamics/1(Plant)
  Env3/1 -> Aerodynamics/2(EnvData)  "ENV"
  Env1/1 -> Bus Selector/1  "ENV"
  Bus Selector/1 -> [F_gravity]  "<Fg>"
  [F_aero] -> Add/1
  [F_thrust] -> Add/2
  [F_gravity] -> Add/3
  [M_aero] -> Add1/1
  [M_thrust] -> Add1/2
  Compare To Constant/1 -> [launched]
  [launched] -> Product/1
  Product/1 -> Time Varying Parameters/1(t)
  Add/1 -> Product1/1
  Add1/1 -> Product2/2
  [launched] -> Product2/1, Product1/2
  Add Constant/1 -> Product/2
  Constant1/1 -> Add2/2
  Add2/1 -> Bus Creator/15  "CG_nose"
  6DOF Equations of Motion/13(q_be) -> [q_be]
  [q_be] -> Bus Creator/19  "q_be"
  6DOF Equations of Motion/8(alpha_total) -> [alpha_total]
  [alpha_total] -> Bus Creator/11  "alpha_total"

== system STEVE_Simulation_6DOF/Visualization/Stop Conditions ==
  In1 : Inport
  AND : Logic  IconShape=distinctive  AllPortsSameDT=off  OutDataTypeStr=boolean
  Abs : Abs  SaturateOnIntegerOverflow=off
  Abs1 : Abs  SaturateOnIntegerOverflow=off
  Bus Selector : BusSelector  OutputSignals=alpha,beta
  Clock : Clock
  Compare To Constant : simulink/Logic and Bit Operations/Compare To Constant  relop=>=  const=40  OutDataTypeStr=boolean
  Compare To Constant1 : simulink/Logic and Bit Operations/Compare To Constant  relop=>=  const=warm_up_time  OutDataTypeStr=boolean
  Max : MinMax  Function=max  Inputs=2
  Radians to Degrees : simulink_extras/Transformations/Radians to Degrees
  Stop Simulation : Stop
  wires:
  In1/1 -> Bus Selector/1
  Bus Selector/1 -> Abs/1  "<alpha>"
  Bus Selector/2 -> Abs1/1  "<beta>"
  Max/1 -> Radians to Degrees/1
  Radians to Degrees/1 -> Compare To Constant/1
  Compare To Constant/1 -> AND/2
  Abs/1 -> Max/1
  Abs1/1 -> Max/2
  AND/1 -> Stop Simulation/1
  Clock/1 -> Compare To Constant1/1
  Compare To Constant1/1 -> AND/1

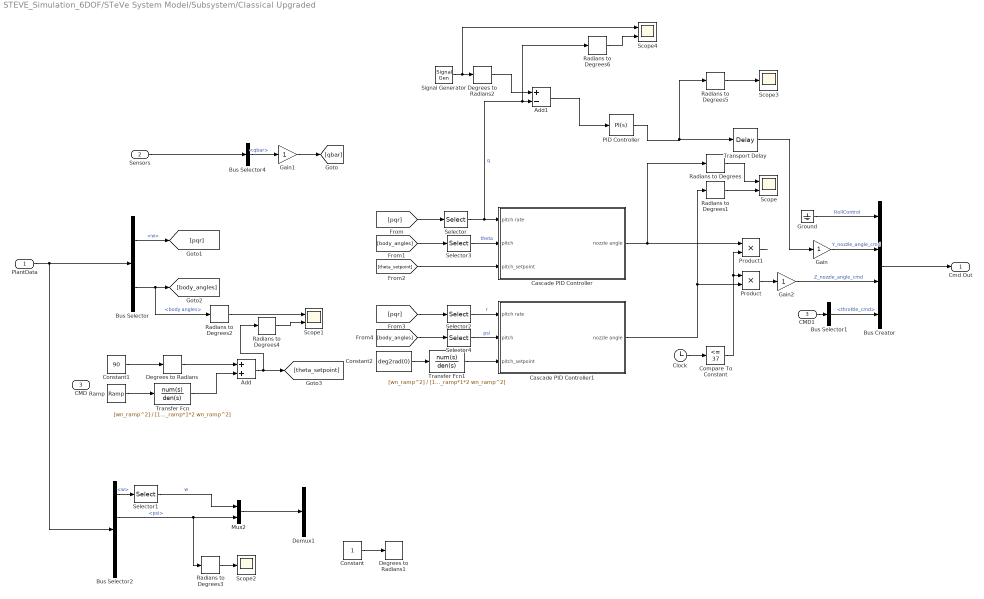
== system STEVE_Simulation_6DOF/STeVe System Model/Subsystem/Classical Upgraded ==
  PlantData : Inport
  Sensors : Inport  Port=2
  CMD : Inport  Port=3
  Add : Sum
  Add1 : Sum  Inputs=+-
  Bus Creator : BusCreator  Inputs=4
  Bus Selector : BusSelector  OutputSignals=w,body angles
  Bus Selector1 : BusSelector  OutputSignals=throttle_cmd
  Bus Selector2 : BusSelector  OutputSignals=w,body angles.psi,Ve,V_air
  Bus Selector4 : BusSelector  OutputSignals=qbar
  CMD1 : InportShadow  Port=3
  Cascade PID Controller : Subsystem
  Cascade PID Controller1 : Subsystem
  Clock : Clock
  Compare To Constant : simulink/Logic and Bit Operations/Compare To Constant  relop=<=  const=37  OutDataTypeStr=boolean
  Constant : Constant
  Constant1 : Constant  Value=90
  Constant2 : Constant  Value=deg2rad(0)
  Degrees to Radians : simulink_extras/Transformations/Degrees to Radians
  Degrees to Radians1 : simulink_extras/Transformations/Degrees to Radians
  Degrees to Radians2 : simulink_extras/Transformations/Degrees to Radians
  Demux1 : Demux  Outputs=2
  Gain : Gain
  Gain1 : Gain
  Gain2 : Gain
  Ground : Ground
  Mux2 : Mux  Inputs=2
  PID Controller : slpidlib/PID Controller  Controller=PI  Form=Parallel  TimeDomain=Continuous-time  UseExternalTs=off  SampleTime=-1  IntegratorMethod=Forward Euler  FilterMethod=Forward Euler  ControllerParametersSource=internal  P=1.8265  I=14.0169  UseKiTs=off  D=0  UseExternalDerivativeSource=off  N=100  UseFilter=on  TunerSelectOption=Transfer Function Based (PID Tuner App)  InitialConditionSource=internal  InitialConditionForIntegrator=0  InitialConditionForFilter=0  DifferentiatorICPrevScaledInput=0  ExternalReset=none  TrackingMode=off  Kt=1  LimitOutput=off  SatLimitsSource=internal  UpperSaturationLimit=inf  LowerSaturationLimit=-inf  LinearizeAsGain=on  AntiWindupMode=none  Kb=1  LimitIntegrator=off  UpperIntegratorSaturationLimit=inf  LowerIntegratorSaturationLimit=-inf  POutMin=[]  POutMax=[]  IOutMin=[]  IOutMax=[]  DOutMin=[]  DOutMax=[]  NOutMin=[]  NOutMax=[]  SumOutMin=[]  SumOutMax=[]  SaturationOutMin=[]  SaturationOutMax=[]  PParamMin=[]  PParamMax=[]  IParamMin=[]  IParamMax=[]  DParamMin=[]  DParamMax=[]  NParamMin=[]  NParamMax=[]  KbParamMin=[]  KbParamMax=[]  KtParamMin=[]  KtParamMax=[]  KbOutMin=[]  KbOutMax=[]  KtOutMin=[]  KtOutMax=[]  IntegratorOutMin=[]  IntegratorOutMax=[]  FilterOutMin=[]  FilterOutMax=[]  SumI1OutMin=[]  SumI1OutMax=[]  SumI2OutMin=[]  SumI2OutMax=[]  SumI3OutMin=[]  SumI3OutMax=[]  SumI4OutMin=[]  SumI4OutMax=[]  SumDOutMin=[]  SumDOutMax=[]  DifferentiatorOutMin=[]  DifferentiatorOutMax=[]  FilterDiffOutCoefMin=[]  FilterDiffOutCoefMax=[]  ReciprocalOutMin=[]  ReciprocalOutMax=[]  SumDenOutMin=[]  SumDenOutMax=[]  SumNumOutMin=[]  SumNumOutMax=[]  DivideOutMin=[]  DivideOutMax=[]  UdiffTsProdOutMin=[]  UdiffTsProdOutMax=[]  NTsProdOutMin=[]  NTsProdOutMax=[]  UintegralTsProdOutMin=[]  UintegralTsProdOutMax=[]  UngainTsProdOutMin=[]  UngainTsProdOutMax=[]  ClampingZeroOutDataTypeStr=Inherit: Inherit via back propagation  ClampingZeroOutMin=[]  ClampingZeroOutMax=[]  FilterDenConstantOutDataTypeStr=Inherit: Inherit via back propagation  FilterDenConstantOutMin=[]  FilterDenConstantOutMax=[]  PCopyOutDataTypeStr=Inherit: Inherit via back propagation  PCopyOutMin=[]  PCopyOutMax=[]  NCopyOutDataTypeStr=Inherit: Inherit via back propagation  NCopyOutMin=[]  NCopyOutMax=[]  IntegratorContinuousStateAttributes=''  IntegratorStateMustResolveToSignalObject=off  IntegratorRTWStateStorageClass=Auto  FilterContinuousStateAttributes=''  FilterStateMustResolveToSignalObject=off  FilterRTWStateStorageClass=Auto  ParallelPVariant=InternalParameters  IdealPVariant=Disabled  IVariant=InternalParameters  DVariant=Disabled  IntegratorVariant=Continuous  SatVariant=Disabled  AWVariant=Passthrough  PCopyVariant=Disabled  TRVariant=Disabled  FdbkBlocksVariant=Forward  IdealPFdbkVariant=Disabled  SatFdbkVariant=Disabled  DerivativeFilterVariant=Disabled  NVariant=Disabled  NCopyVariant=Disabled_SignalSpec  FilterICVariant=Disabled  IntegratorICVariant=InternalICs  ExternalResetVariant=Disabled  TRSumVariant=Passthrough  SumFdbkVariant=Disabled  SumVariant=Sum_PI  TsampFilterVariant=InternalTs  TsampNgainVariant=Passthrough  TsampIntegralVariant=Disabled_SignalSpec  ExternalSaturationOutDataTypeStr=Inherit: Same as second input  DerivativeSourceVariant=Disabled  PreIntVariant=InternalPreInt
  Product : Product
  Product1 : Product
  Radians to Degrees{,1..6} (7 alike) : simulink_extras/Transformations/Radians to Degrees
  Ramp : simulink/Sources/Ramp  slope=-(10/60)*pi/180  start=0  InitialOutput=0
  Scope : Scope  NumInputPorts=2
      settings: ActiveDisplayYMinimum=-2.0223368539006419  ActiveDisplayYMaximum=0.30837107460030577  DataLoggingVariableName=ScopeData10
  Scope1 : Scope  NumInputPorts=2
      settings: ActiveDisplayYMinimum=-85.342848172773913  ActiveDisplayYMaximum=210.22972215938358  DataLoggingVariableName=ScopeData11
  Scope2 : Scope
      settings: ActiveDisplayYMinimum=-18.362797933212903  ActiveDisplayYMaximum=16.52585265642092  DataLoggingVariableName=ScopeData7
  Scope3 : Scope
      settings: ActiveDisplayYMinimum=-2535.4711139327528  ActiveDisplayYMaximum=531.06890360245575  DataLoggingVariableName=ScopeData12
  Scope4 : Scope  NumInputPorts=2
      settings: ActiveDisplayYMinimum=-83.658192950020577  ActiveDisplayYMaximum=117.69725689081616  DataLoggingVariableName=ScopeData13
  Selector : Selector  InputPortWidth=3  IndexOptions=Index vector (dialog)  Indices=[2]  OutputSizes=1
  Selector1 : Selector  InputPortWidth=3  IndexOptions=Index vector (dialog)  Indices=[3]  OutputSizes=1
  Selector2 : Selector  InputPortWidth=3  IndexOptions=Index vector (dialog)  Indices=[3]  OutputSizes=1
  Selector3 : Selector  InputPortWidth=3  IndexOptions=Index vector (dialog)  Indices=[2]  OutputSizes=1
  Selector4 : Selector  InputPortWidth=3  IndexOptions=Index vector (dialog)  Indices=[3]  OutputSizes=1
  Signal Generator : SignalGenerator  Amplitude=10  Frequency=0.5
  Transfer Fcn : TransferFcn  Numerator=[wn_ramp^2]  Denominator=[1 wn_ramp*1*2 wn_ramp^2]
  Transfer Fcn1 : TransferFcn  Numerator=[wn_ramp^2]  Denominator=[1 wn_ramp*1*2 wn_ramp^2]
  Transport Delay : TransportDelay  DelayTime=0.05
  Cmd Out : Outport
  wires:
  Gain/1 -> Bus Creator/2  "Y_nozzle_angle_cmd"
  Ground/1 -> Bus Creator/1  "RollControl"
  Bus Creator/1 -> Cmd Out/1
  CMD1/1 -> Bus Selector1/1
  Bus Selector1/1 -> Bus Creator/4  "<throttle_cmd>"
  Ramp/1 -> Transfer Fcn/1
  Constant1/1 -> Degrees to Radians/1
  Selector/1 -> Radians to Degrees6/1, Add1/2, Cascade PID Controller/1(pitch rate)  "q"
  Sensors/1 -> Bus Selector4/1
  Bus Selector4/1 -> Gain1/1  "<qbar>"
  PlantData/1 -> Bus Selector2/1, Bus Selector/1
  Mux2/1 -> Demux1/1
  Bus Selector2/1 -> Selector1/1  "<w>"
  Selector1/1 -> Mux2/1  "w"
  Bus Selector2/2 -> Radians to Degrees3/1, Mux2/2  "<psi>"
  Gain1/1 -> [qbar]
  Constant/1 -> Degrees to Radians1/1
  Degrees to Radians/1 -> Add/1
  Gain2/1 -> Bus Creator/3  "Z_nozzle_angle_cmd"
  Radians to Degrees3/1 -> Scope2/1
  Transfer Fcn/1 -> Add/2
  Cascade PID Controller/1(nozzle angle) -> Product1/1, Radians to Degrees/1
  Bus Selector/1 -> [pqr]  "<w>"
  Bus Selector/2 -> Radians to Degrees2/1, [body_angles]  "<body angles>"
  [pqr] -> Selector/1
  [body_angles] -> Selector3/1
  Selector3/1 -> Cascade PID Controller/2(pitch)  "theta"
  Add/1 -> Radians to Degrees4/1, [theta_setpoint]
  [theta_setpoint] -> Cascade PID Controller/3(pitch_setpoint)
  [body_angles] -> Selector4/1
  [pqr] -> Selector2/1
  Selector4/1 -> Cascade PID Controller1/2(pitch)  "psi"
  Selector2/1 -> Cascade PID Controller1/1(pitch rate)  "r"
  Constant2/1 -> Transfer Fcn1/1
  Cascade PID Controller1/1(nozzle angle) -> Radians to Degrees1/1, Product/2
  Radians to Degrees/1 -> Scope/1
  Radians to Degrees1/1 -> Scope/2
  Transfer Fcn1/1 -> Cascade PID Controller1/3(pitch_setpoint)
  Radians to Degrees2/1 -> Scope1/1
  Radians to Degrees4/1 -> Scope1/2
  Product/1 -> Gain2/1
  Product1/1 -> ?
  Clock/1 -> Compare To Constant/1
  Compare To Constant/1 -> Product1/2, Product/1
  PID Controller/1 -> Radians to Degrees5/1, Transport Delay/1
  Radians to Degrees5/1 -> Scope3/1
  Add1/1 -> PID Controller/1
  Signal Generator/1 -> Scope4/1, Degrees to Radians2/1
  Degrees to Radians2/1 -> Add1/1
  Radians to Degrees6/1 -> Scope4/2
  Transport Delay/1 -> Gain/1

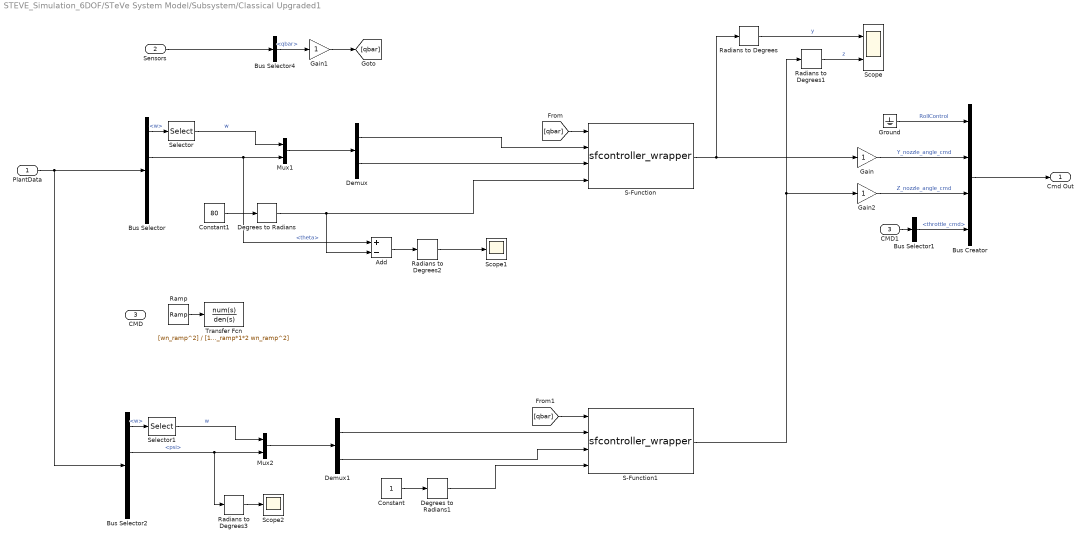
== system STEVE_Simulation_6DOF/STeVe System Model/Subsystem/Classical Upgraded1 ==
  PlantData : Inport
  Sensors : Inport  Port=2
  CMD : Inport  Port=3
  Add : Sum  Inputs=+-
  Bus Creator : BusCreator  Inputs=4
  Bus Selector : BusSelector  OutputSignals=w,body angles.theta,Ve,V_air
  Bus Selector1 : BusSelector  OutputSignals=throttle_cmd
  Bus Selector2 : BusSelector  OutputSignals=w,body angles.psi,Ve,V_air
  Bus Selector4 : BusSelector  OutputSignals=qbar
  CMD1 : InportShadow  Port=3
  Constant : Constant
  Constant1 : Constant  Value=80
  Degrees to Radians : simulink_extras/Transformations/Degrees to Radians
  Degrees to Radians1 : simulink_extras/Transformations/Degrees to Radians
  Demux : Demux  Outputs=2
  Demux1 : Demux  Outputs=2
  Gain : Gain
  Gain1 : Gain
  Gain2 : Gain
  Ground : Ground
  Mux1 : Mux  Inputs=2
  Mux2 : Mux  Inputs=2
  Radians to Degrees{,1..3} (4 alike) : simulink_extras/Transformations/Radians to Degrees
  Ramp : simulink/Sources/Ramp  slope=-(10/60)*pi/180  start=0  InitialOutput=0
  S-Function : S-Function  FunctionName=sfcontroller_wrapper  Parameters=1/200  SFunctionDeploymentMode=off  EnableBusSupport=off
  S-Function1 : S-Function  FunctionName=sfcontroller_wrapper  Parameters=1/200  SFunctionDeploymentMode=off  EnableBusSupport=off
  Scope : Scope  NumInputPorts=2
      settings: ActiveDisplayYMinimum=-4.2204024773841731  ActiveDisplayYMaximum=1.0481503715635636
  Scope1 : Scope
      settings: ActiveDisplayYMinimum=-9.8558967366890791  ActiveDisplayYMaximum=9.0134421432183061  DataLoggingVariableName=ScopeData6
  Scope2 : Scope
      settings: ActiveDisplayYMinimum=-18.362797933212903  ActiveDisplayYMaximum=16.52585265642092  DataLoggingVariableName=ScopeData7
  Selector : Selector  InputPortWidth=3  IndexOptions=Index vector (dialog)  Indices=[2]  OutputSizes=1
  Selector1 : Selector  InputPortWidth=3  IndexOptions=Index vector (dialog)  Indices=[3]  OutputSizes=1
  Transfer Fcn : TransferFcn  Numerator=[wn_ramp^2]  Denominator=[1 wn_ramp*1*2 wn_ramp^2]
  Cmd Out : Outport
  wires:
  Bus Selector/1 -> Selector/1  "<w>"
  S-Function1/1 -> Radians to Degrees1/1, Gain2/1
  Gain/1 -> Bus Creator/2  "Y_nozzle_angle_cmd"
  Ground/1 -> Bus Creator/1  "RollControl"
  Bus Creator/1 -> Cmd Out/1
  CMD1/1 -> Bus Selector1/1
  Bus Selector1/1 -> Bus Creator/4  "<throttle_cmd>"
  Bus Selector/2 -> Add/1, Mux1/2  "<theta>"
  Ramp/1 -> Transfer Fcn/1
  Constant1/1 -> Degrees to Radians/1
  Mux1/1 -> Demux/1
  Demux/1 -> S-Function/2
  Demux/2 -> S-Function/3
  Selector/1 -> Mux1/1  "w"
  Sensors/1 -> Bus Selector4/1
  Bus Selector4/1 -> Gain1/1  "<qbar>"
  S-Function/1 -> Radians to Degrees/1, Gain/1
  Demux1/2 -> S-Function1/3
  PlantData/1 -> Bus Selector2/1, Bus Selector/1
  Mux2/1 -> Demux1/1
  Bus Selector2/1 -> Selector1/1  "<w>"
  Selector1/1 -> Mux2/1  "w"
  Bus Selector2/2 -> Radians to Degrees3/1, Mux2/2  "<psi>"
  Demux1/1 -> S-Function1/2
  Gain1/1 -> [qbar]
  [qbar] -> S-Function/1
  [qbar] -> S-Function1/1
  Constant/1 -> Degrees to Radians1/1
  Degrees to Radians/1 -> Add/2, S-Function/4
  Radians to Degrees/1 -> Scope/1  "y"
  Radians to Degrees1/1 -> Scope/2  "z"
  Gain2/1 -> Bus Creator/3  "Z_nozzle_angle_cmd"
  Add/1 -> Radians to Degrees2/1
  Radians to Degrees2/1 -> Scope1/1
  Degrees to Radians1/1 -> S-Function1/4
  Radians to Degrees3/1 -> Scope2/1

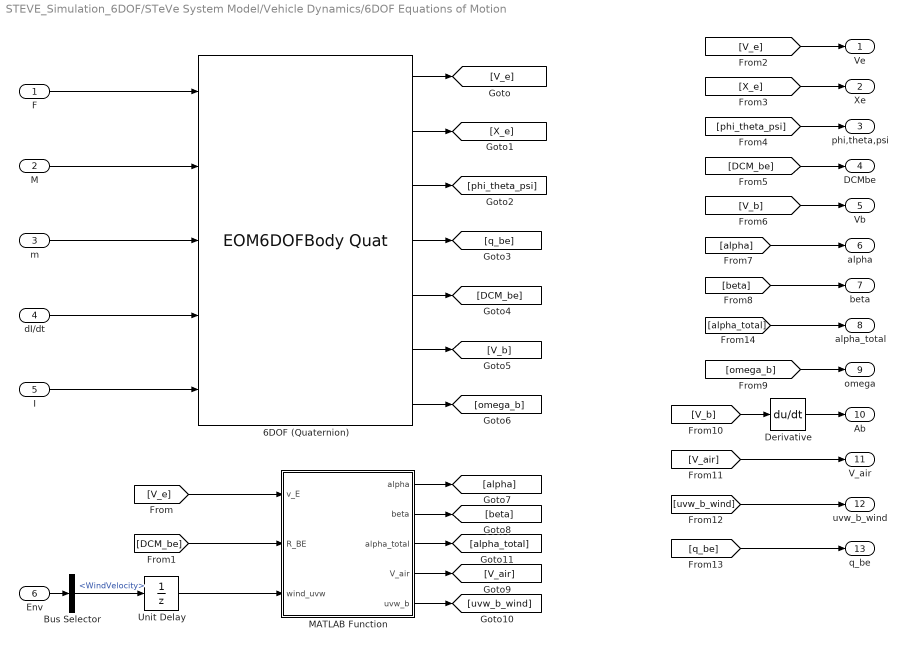
== system STEVE_Simulation_6DOF/STeVe System Model/Vehicle Dynamics/6DOF Equations of Motion ==
  F : Inport
  M : Inport  Port=2
  m : Inport  Port=3
  dI/dt : Inport  Port=4
  I : Inport  Port=5
  Env : Inport  Port=6
  6DOF (Quaternion) : EOM6DOFBodyQuat  mtype=Custom Variable  Vm_0=[0.01 0 0]  eul_0=euler_0  Vm_statename={'U','v','w'}  xme_statename={'Xe','Ye','Ze'}  pm_statename={'p','q','r'}  quat_statename={'qr','qi','qj','qk'}
  Bus Selector : BusSelector  OutputSignals=WindVelocity
  Derivative : Derivative
  MATLAB Function : MATLAB Function  TreatAsAtomicUnit=on
  Unit Delay : UnitDelay  SampleTime=-1  HasFrameUpgradeWarning=on
  Ve : Outport
  Xe : Outport  Port=2
  phi,theta,psi : Outport  Port=3
  DCMbe : Outport  Port=4
  Vb : Outport  Port=5
  alpha : Outport  Port=6
  beta : Outport  Port=7
  alpha_total : Outport  Port=8
  omega : Outport  Port=9
  Ab : Outport  Port=10
  V_air : Outport  Port=11
  uvw_b_wind : Outport  Port=12
  q_be : Outport  Port=13
  wires:
  F/1 -> 6DOF (Quaternion)/1
  M/1 -> 6DOF (Quaternion)/2
  [phi_theta_psi] -> phi,theta,psi/1
  [omega_b] -> omega/1
  [DCM_be] -> DCMbe/1
  [X_e] -> Xe/1
  [V_b] -> Vb/1
  [V_e] -> Ve/1
  Derivative/1 -> Ab/1
  I/1 -> 6DOF (Quaternion)/5
  dI/dt/1 -> 6DOF (Quaternion)/4
  Env/1 -> Bus Selector/1
  Bus Selector/1 -> Unit Delay/1  "<WindVelocity>"
  m/1 -> 6DOF (Quaternion)/3
  6DOF (Quaternion)/1 -> [V_e]
  6DOF (Quaternion)/2 -> [X_e]
  6DOF (Quaternion)/3 -> [phi_theta_psi]
  6DOF (Quaternion)/4 -> [q_be]
  6DOF (Quaternion)/5 -> [DCM_be]
  6DOF (Quaternion)/6 -> [V_b]
  6DOF (Quaternion)/7 -> [omega_b]
  [V_e] -> MATLAB Function/1(v_E)
  [DCM_be] -> MATLAB Function/2(R_BE)
  MATLAB Function/1(alpha) -> [alpha]
  MATLAB Function/2(beta) -> [beta]
  MATLAB Function/4(V_air) -> [V_air]
  MATLAB Function/5(uvw_b) -> [uvw_b_wind]
  [alpha] -> alpha/1
  [beta] -> beta/1
  [V_b] -> Derivative/1
  [V_air] -> V_air/1
  [uvw_b_wind] -> uvw_b_wind/1
  [q_be] -> q_be/1
  Unit Delay/1 -> MATLAB Function/3(wind_uvw)
  MATLAB Function/3(alpha_total) -> [alpha_total]
  [alpha_total] -> alpha_total/1

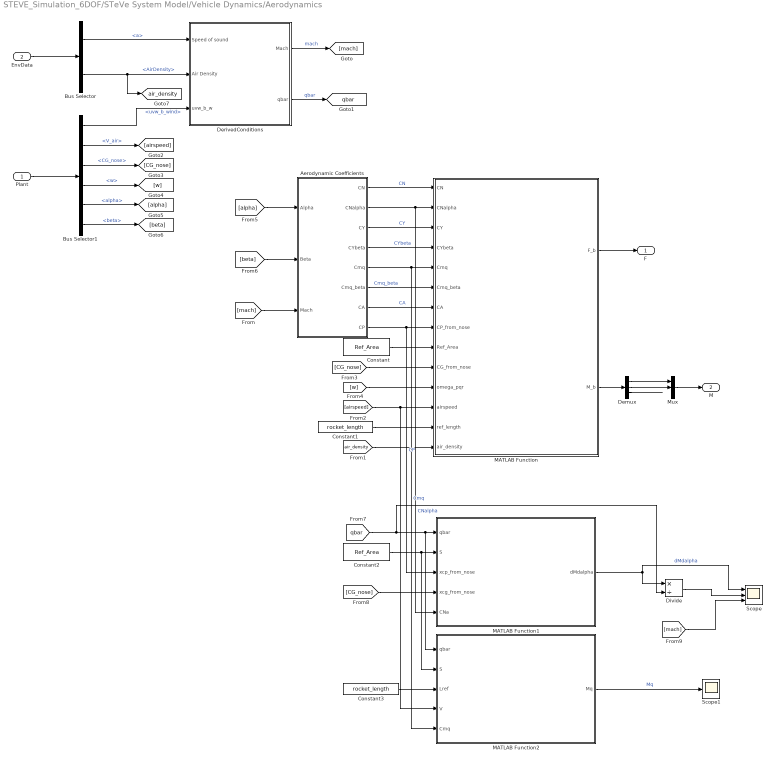
== system STEVE_Simulation_6DOF/STeVe System Model/Vehicle Dynamics/Aerodynamics ==
  Plant : Inport
  EnvData : Inport  Port=2
  "Aerodynamic Coefficients " : Subsystem
  Bus Selector : BusSelector  OutputSignals=a,AirDensity
  Bus Selector1 : BusSelector  OutputSignals=uvw_b_wind,V_air,CG_nose,w,alpha,beta
  Constant : Constant  Value=Ref_Area  VectorParams1D=off
  Constant1 : Constant  Value=rocket_length
  Constant2 : Constant  Value=Ref_Area  VectorParams1D=off
  Constant3 : Constant  Value=rocket_length
  Demux : Demux  Outputs=3
  DerivedConditions : Subsystem
  Divide : Product  Inputs=*/
  MATLAB Function : MATLAB Function  TreatAsAtomicUnit=on
  MATLAB Function1 : MATLAB Function  TreatAsAtomicUnit=on
  MATLAB Function2 : MATLAB Function  TreatAsAtomicUnit=on
  Mux : Mux  Inputs=3
  Scope : Scope  NumInputPorts=3
      settings: ActiveDisplayYMinimum=-20269.526617708132  ActiveDisplayYMaximum=182425.7406044511  DataLoggingVariableName=ScopeData8
  Scope1 : Scope
      settings: ActiveDisplayYMinimum=-5298.2755475796475  ActiveDisplayYMaximum=588.69728306440516  DataLoggingVariableName=ScopeData9
  F : Outport
  M : Outport  Port=2
  tag scope: air_density=global, qbar=global
  wires:
  Plant/1 -> Bus Selector1/1
  EnvData/1 -> Bus Selector/1
  Bus Selector/2 -> [air_density], DerivedConditions/2(Air Density)  "<AirDensity>"
  Bus Selector/1 -> DerivedConditions/1(Speed of sound)  "<a>"
  DerivedConditions/1(Mach) -> [mach]  "mach"
  DerivedConditions/2(qbar) -> [qbar]  "qbar"
  [mach] -> "Aerodynamic Coefficients "/3(Mach)
  MATLAB Function/1(F_b) -> F/1
  MATLAB Function/2(M_b) -> Demux/1
  Bus Selector1/2 -> [airspeed]  "<V_air>"
  Bus Selector1/1 -> DerivedConditions/3(uvw_b_w)  "<uvw_b_wind>"
  Bus Selector1/3 -> [CG_nose]  "<CG_nose>"
  Bus Selector1/4 -> [w]  "<w>"
  Bus Selector1/5 -> [alpha]  "<alpha>"
  Bus Selector1/6 -> [beta]  "<beta>"
  [alpha] -> "Aerodynamic Coefficients "/1(Alpha)
  [beta] -> "Aerodynamic Coefficients "/2(Beta)
  "Aerodynamic Coefficients "/1(CN) -> MATLAB Function/1(CN)  "CN"
  "Aerodynamic Coefficients "/2(CNalpha) -> MATLAB Function1/5(CNa), MATLAB Function/2(CNalpha)  "CNalpha"
  "Aerodynamic Coefficients "/3(CY) -> MATLAB Function/3(CY)  "CY"
  "Aerodynamic Coefficients "/4(CYbeta) -> MATLAB Function/4(CYbeta)  "CYbeta"
  "Aerodynamic Coefficients "/5(Cmq) -> MATLAB Function2/5(Cmq), MATLAB Function/5(Cmq)  "Cmq"
  "Aerodynamic Coefficients "/6(Cmq_beta) -> MATLAB Function/6(Cmq_beta)  "Cmq_beta"
  "Aerodynamic Coefficients "/7(CA) -> MATLAB Function/7(CA)  "CA"
  "Aerodynamic Coefficients "/8(CP) -> MATLAB Function1/3(xcp_from_nose), MATLAB Function/8(CP_from_nose)  "CP"
  Constant/1 -> MATLAB Function/9(Ref_Area)
  [CG_nose] -> MATLAB Function/10(CG_from_nose)
  [w] -> MATLAB Function/11(omega_pqr)
  [airspeed] -> MATLAB Function2/4(V), MATLAB Function/12(airspeed)
  [air_density] -> MATLAB Function/14(air_density)
  Constant1/1 -> MATLAB Function/13(ref_length)
  Demux/2 -> Mux/2
  Mux/1 -> M/1
  Demux/1 -> Mux/1
  Demux/3 -> ?
  [qbar] -> Divide/2, MATLAB Function2/1(qbar), MATLAB Function1/1(qbar)
  Constant2/1 -> MATLAB Function2/2(S), MATLAB Function1/2(S)
  [CG_nose] -> MATLAB Function1/4(xcg_from_nose)
  MATLAB Function1/1(dMdalpha) -> Divide/1, Scope/1  "dMdalpha"
  Divide/1 -> Scope/2
  [mach] -> Scope/3
  Constant3/1 -> MATLAB Function2/3(Lref)
  MATLAB Function2/1(Mq) -> Scope1/1  "Mq"

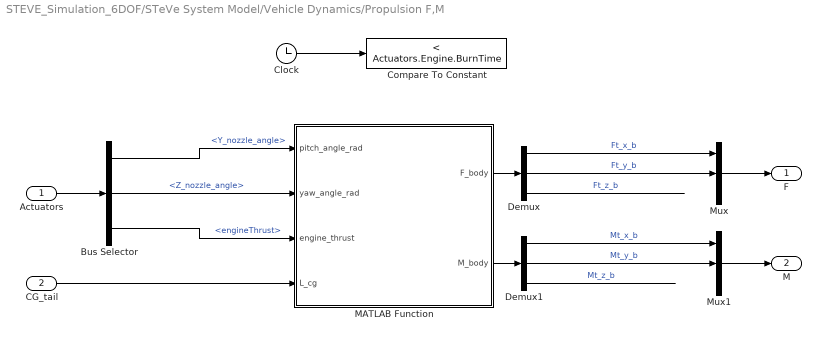
== system STEVE_Simulation_6DOF/STeVe System Model/Vehicle Dynamics/Propulsion F,M ==
  Actuators : Inport
  CG_tail : Inport  Port=2
  Bus Selector : BusSelector  OutputSignals=Y_nozzle_angle,Z_nozzle_angle,engineThrust
  Clock : Clock
  Compare To Constant : simulink/Logic and Bit Operations/Compare To Constant  relop=<  const=Actuators.Engine.BurnTime  OutDataTypeStr=boolean
  Demux : Demux  Outputs=3
  Demux1 : Demux  Outputs=3
  MATLAB Function : MATLAB Function  TreatAsAtomicUnit=on
  Mux : Mux  Inputs=3
  Mux1 : Mux  Inputs=3
  F : Outport
  M : Outport  Port=2
  wires:
  Actuators/1 -> Bus Selector/1
  Bus Selector/1 -> MATLAB Function/1(pitch_angle_rad)  "<Y_nozzle_angle>"
  Bus Selector/3 -> MATLAB Function/3(engine_thrust)  "<engineThrust>"
  Demux/3 -> ?  "Ft_z_b"
  Mux/1 -> F/1
  Mux1/1 -> M/1
  Demux1/1 -> Mux1/1  "Mt_x_b"
  Demux1/3 -> ?  "Mt_z_b"
  CG_tail/1 -> MATLAB Function/4(L_cg)
  Clock/1 -> Compare To Constant/1
  Demux/1 -> Mux/1  "Ft_x_b"
  Bus Selector/2 -> MATLAB Function/2(yaw_angle_rad)  "<Z_nozzle_angle>"
  MATLAB Function/1(F_body) -> Demux/1
  MATLAB Function/2(M_body) -> Demux1/1
  Demux1/2 -> Mux1/2  "Mt_y_b"
  Demux/2 -> Mux/2  "Ft_y_b"

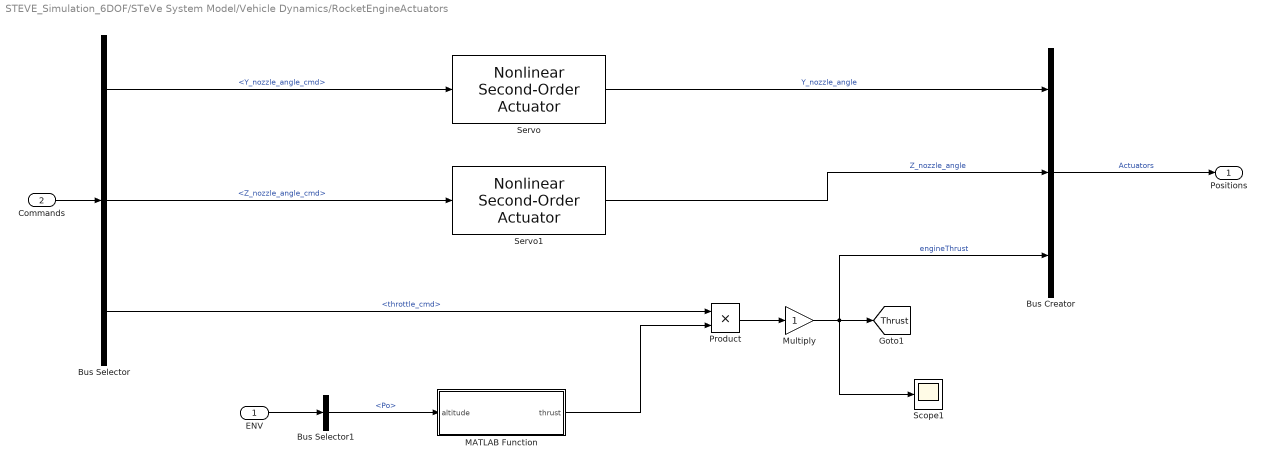
== system STEVE_Simulation_6DOF/STeVe System Model/Vehicle Dynamics/RocketEngineActuators ==
  ENV : Inport
  Commands : Inport  Port=2
  Bus Creator : BusCreator  Inputs=3
  Bus Selector : BusSelector  OutputSignals=Y_nozzle_angle_cmd,Z_nozzle_angle_cmd,throttle_cmd
  Bus Selector1 : BusSelector  OutputSignals=Po
  MATLAB Function : MATLAB Function  TreatAsAtomicUnit=on
  Multiply : Gain
  Product : Product
  Scope1 : Scope
      settings: ActiveDisplayYMinimum=-3298.6854275413052  ActiveDisplayYMaximum=31070.467018460706  DataLoggingVariableName=ScopeData2
  Servo : aerolibactuator/Nonlinear Second-Order Actuator  wn_fin=62  z_fin=0.5858  fin_max=10*pi/180  fin_min=-10*pi/180  fin_maxrate=(1000*pi/180)  fin_act_0=0  fin_act_vel=0
  Servo1 : aerolibactuator/Nonlinear Second-Order Actuator  wn_fin=62  z_fin=0.5858  fin_max=10*pi/180  fin_min=-10*pi/180  fin_maxrate=(1000*pi/180)  fin_act_0=0  fin_act_vel=0
  Positions : Outport
  tag scope: Thrust=global
  wires:
  Commands/1 -> Bus Selector/1
  Bus Creator/1 -> Positions/1  "Actuators"
  Bus Selector/3 -> Product/1  "<throttle_cmd>"
  ENV/1 -> Bus Selector1/1
  Bus Selector1/1 -> MATLAB Function/1(altitude)  "<Po>"
  MATLAB Function/1(thrust) -> Product/2
  Product/1 -> Multiply/1
  Bus Selector/1 -> Servo/1  "<Y_nozzle_angle_cmd>"
  Multiply/1 -> Bus Creator/3, [Thrust], Scope1/1  "engineThrust"
  Servo/1 -> Bus Creator/1  "Y_nozzle_angle"
  Servo1/1 -> Bus Creator/2  "Z_nozzle_angle"
  Bus Selector/2 -> Servo1/1  "<Z_nozzle_angle_cmd>"

== system STEVE_Simulation_6DOF/STeVe System Model/Vehicle Dynamics/Time Varying Parameters ==
  t : Inport
  Direct Lookup Table (n-D) : LookupNDDirect  NumberOfTableDimensions=3  InputsSelectThisObjectFromTable=2-D Matrix  Table=PrelookupData.Tables.InertialTensor  DiagnosticForOutOfRangeInput=None  TableDataTypeStr=double
  Direct Lookup Table (n-D)1 : LookupNDDirect  NumberOfTableDimensions=3  InputsSelectThisObjectFromTable=2-D Matrix  Table=PrelookupData.Tables.dInertialTensor  DiagnosticForOutOfRangeInput=None  TableDataTypeStr=double
  Lookup_COM_X : Interpolation_n-D  NumberOfTableDimensions=1  Table=PrelookupData.Tables.COM_X  ExtrapMethod=Clip  DiagnosticForOutOfRangeInput=Warning  RequireIndexFractionAsBus=on  InternalRulePriority=Speed
      settings: InputPortMap=u0
  Lookup_Mass : Interpolation_n-D  NumberOfTableDimensions=1  Table=PrelookupData.Tables.Mass  ExtrapMethod=Clip  DiagnosticForOutOfRangeInput=Warning  RequireIndexFractionAsBus=on  OutDataTypeStr=double  InternalRulePriority=Speed  TableDataTypeStr=Inherit: Inherit from 'Table data'
      settings: InputPortMap=u0
  Prelookup : PreLookup  BreakpointsData=PrelookupData.Breakpoints.Index  OutputSelection=Index and fraction as bus  IndexSearchMethod=Evenly spaced points
  TimeToIndex : Subsystem
  dIdt_Tensor(3x3) : Outport
  MOI_Tensor(3x3) : Outport  Port=2
  mass : Outport  Port=3
  COM_X_Tail : Outport  Port=4
  wires:
  Lookup_Mass/1 -> mass/1  "mass"
  t/1 -> TimeToIndex/1(t)
  Lookup_COM_X/1 -> COM_X_Tail/1  "CG_from_tail"
  Direct Lookup Table (n-D)/1 -> MOI_Tensor(3x3)/1
  Direct Lookup Table (n-D)1/1 -> dIdt_Tensor(3x3)/1
  Prelookup/1 -> Lookup_Mass/1, Lookup_COM_X/1
  TimeToIndex/1(Index) -> Direct Lookup Table (n-D)/1, Direct Lookup Table (n-D)1/1, Prelookup/1

== system STEVE_Simulation_6DOF/STeVe System Model/Subsystem/Classical Upgraded/Cascade PID Controller ==
  pitch rate : Inport
  pitch : Inport  Port=2
  pitch_setpoint : Inport  Port=3
  Add : Sum  Inputs=-+
  Add1 : Sum  Inputs=-+
  Pitch Controller : slpidlib/PID Controller  Controller=PI  Form=Parallel  TimeDomain=Discrete-time  UseExternalTs=off  SampleTime=Ts_outer  IntegratorMethod=Forward Euler  FilterMethod=Forward Euler  ControllerParametersSource=internal  P=C_outer_maxQ_d_Kp  I=C_outer_maxQ_d_Ki  UseKiTs=off  D=0.164283893804061  UseExternalDerivativeSource=off  N=4651.32243718652  UseFilter=on  TunerSelectOption=Transfer Function Based (PID Tuner App)  InitialConditionSource=internal  InitialConditionForIntegrator=0  InitialConditionForFilter=0  DifferentiatorICPrevScaledInput=0  ExternalReset=none  TrackingMode=off  Kt=1  LimitOutput=off  SatLimitsSource=internal  UpperSaturationLimit=inf  LowerSaturationLimit=-inf  LinearizeAsGain=on  AntiWindupMode=none  Kb=1  LimitIntegrator=off  UpperIntegratorSaturationLimit=inf  LowerIntegratorSaturationLimit=-inf  POutMin=[]  POutMax=[]  IOutMin=[]  IOutMax=[]  DOutMin=[]  DOutMax=[]  NOutMin=[]  NOutMax=[]  SumOutMin=[]  SumOutMax=[]  SaturationOutMin=[]  SaturationOutMax=[]  PParamMin=[]  PParamMax=[]  IParamMin=[]  IParamMax=[]  DParamMin=[]  DParamMax=[]  NParamMin=[]  NParamMax=[]  KbParamMin=[]  KbParamMax=[]  KtParamMin=[]  KtParamMax=[]  KbOutMin=[]  KbOutMax=[]  KtOutMin=[]  KtOutMax=[]  IntegratorOutMin=[]  IntegratorOutMax=[]  FilterOutMin=[]  FilterOutMax=[]  SumI1OutMin=[]  SumI1OutMax=[]  SumI2OutMin=[]  SumI2OutMax=[]  SumI3OutMin=[]  SumI3OutMax=[]  SumI4OutMin=[]  SumI4OutMax=[]  SumDOutMin=[]  SumDOutMax=[]  DifferentiatorOutMin=[]  DifferentiatorOutMax=[]  FilterDiffOutCoefMin=[]  FilterDiffOutCoefMax=[]  ReciprocalOutMin=[]  ReciprocalOutMax=[]  SumDenOutMin=[]  SumDenOutMax=[]  SumNumOutMin=[]  SumNumOutMax=[]  DivideOutMin=[]  DivideOutMax=[]  UdiffTsProdOutMin=[]  UdiffTsProdOutMax=[]  NTsProdOutMin=[]  NTsProdOutMax=[]  UintegralTsProdOutMin=[]  UintegralTsProdOutMax=[]  UngainTsProdOutMin=[]  UngainTsProdOutMax=[]  ClampingZeroOutDataTypeStr=Inherit: Inherit via back propagation  ClampingZeroOutMin=[]  ClampingZeroOutMax=[]  FilterDenConstantOutDataTypeStr=Inherit: Inherit via back propagation  FilterDenConstantOutMin=[]  FilterDenConstantOutMax=[]  PCopyOutDataTypeStr=Inherit: Inherit via back propagation  PCopyOutMin=[]  PCopyOutMax=[]  NCopyOutDataTypeStr=Inherit: Inherit via back propagation  NCopyOutMin=[]  NCopyOutMax=[]  IntegratorContinuousStateAttributes=''  IntegratorStateMustResolveToSignalObject=off  IntegratorRTWStateStorageClass=Auto  FilterContinuousStateAttributes=''  FilterStateMustResolveToSignalObject=off  FilterRTWStateStorageClass=Auto  ParallelPVariant=InternalParameters  IdealPVariant=Disabled  IVariant=InternalParameters  DVariant=Disabled  IntegratorVariant=Discrete  SatVariant=Disabled  AWVariant=Passthrough  PCopyVariant=Disabled  TRVariant=Disabled  FdbkBlocksVariant=Forward  IdealPFdbkVariant=Disabled  SatFdbkVariant=Disabled  DerivativeFilterVariant=Disabled  NVariant=Disabled  NCopyVariant=Disabled_SignalSpec  FilterICVariant=Disabled  IntegratorICVariant=InternalICs  ExternalResetVariant=Disabled  TRSumVariant=Passthrough  SumFdbkVariant=Disabled  SumVariant=Sum_PI  TsampFilterVariant=InternalTs  TsampNgainVariant=Passthrough  TsampIntegralVariant=Disabled_SignalSpec  ExternalSaturationOutDataTypeStr=Inherit: Same as second input  DerivativeSourceVariant=Disabled  PreIntVariant=InternalPreInt
  Pitch Rate Controller : slpidlib/PID Controller  Controller=PI  Form=Parallel  TimeDomain=Discrete-time  UseExternalTs=off  SampleTime=Ts_inner  IntegratorMethod=Forward Euler  FilterMethod=Forward Euler  ControllerParametersSource=internal  P=C_inner_maxQ_d_Kp  I=C_inner_maxQ_d_Ki  UseKiTs=off  D=0.164283893804061  UseExternalDerivativeSource=off  N=4651.32243718652  UseFilter=on  TunerSelectOption=Transfer Function Based (PID Tuner App)  InitialConditionSource=internal  InitialConditionForIntegrator=0  InitialConditionForFilter=0  DifferentiatorICPrevScaledInput=0  ExternalReset=none  TrackingMode=off  Kt=1  LimitOutput=off  SatLimitsSource=internal  UpperSaturationLimit=inf  LowerSaturationLimit=-inf  LinearizeAsGain=on  AntiWindupMode=none  Kb=1  LimitIntegrator=off  UpperIntegratorSaturationLimit=inf  LowerIntegratorSaturationLimit=-inf  POutMin=[]  POutMax=[]  IOutMin=[]  IOutMax=[]  DOutMin=[]  DOutMax=[]  NOutMin=[]  NOutMax=[]  SumOutMin=[]  SumOutMax=[]  SaturationOutMin=[]  SaturationOutMax=[]  PParamMin=[]  PParamMax=[]  IParamMin=[]  IParamMax=[]  DParamMin=[]  DParamMax=[]  NParamMin=[]  NParamMax=[]  KbParamMin=[]  KbParamMax=[]  KtParamMin=[]  KtParamMax=[]  KbOutMin=[]  KbOutMax=[]  KtOutMin=[]  KtOutMax=[]  IntegratorOutMin=[]  IntegratorOutMax=[]  FilterOutMin=[]  FilterOutMax=[]  SumI1OutMin=[]  SumI1OutMax=[]  SumI2OutMin=[]  SumI2OutMax=[]  SumI3OutMin=[]  SumI3OutMax=[]  SumI4OutMin=[]  SumI4OutMax=[]  SumDOutMin=[]  SumDOutMax=[]  DifferentiatorOutMin=[]  DifferentiatorOutMax=[]  FilterDiffOutCoefMin=[]  FilterDiffOutCoefMax=[]  ReciprocalOutMin=[]  ReciprocalOutMax=[]  SumDenOutMin=[]  SumDenOutMax=[]  SumNumOutMin=[]  SumNumOutMax=[]  DivideOutMin=[]  DivideOutMax=[]  UdiffTsProdOutMin=[]  UdiffTsProdOutMax=[]  NTsProdOutMin=[]  NTsProdOutMax=[]  UintegralTsProdOutMin=[]  UintegralTsProdOutMax=[]  UngainTsProdOutMin=[]  UngainTsProdOutMax=[]  ClampingZeroOutDataTypeStr=Inherit: Inherit via back propagation  ClampingZeroOutMin=[]  ClampingZeroOutMax=[]  FilterDenConstantOutDataTypeStr=Inherit: Inherit via back propagation  FilterDenConstantOutMin=[]  FilterDenConstantOutMax=[]  PCopyOutDataTypeStr=Inherit: Inherit via back propagation  PCopyOutMin=[]  PCopyOutMax=[]  NCopyOutDataTypeStr=Inherit: Inherit via back propagation  NCopyOutMin=[]  NCopyOutMax=[]  IntegratorContinuousStateAttributes=''  IntegratorStateMustResolveToSignalObject=off  IntegratorRTWStateStorageClass=Auto  FilterContinuousStateAttributes=''  FilterStateMustResolveToSignalObject=off  FilterRTWStateStorageClass=Auto  ParallelPVariant=InternalParameters  IdealPVariant=Disabled  IVariant=InternalParameters  DVariant=Disabled  IntegratorVariant=Discrete  SatVariant=Disabled  AWVariant=Passthrough  PCopyVariant=Disabled  TRVariant=Disabled  FdbkBlocksVariant=Forward  IdealPFdbkVariant=Disabled  SatFdbkVariant=Disabled  DerivativeFilterVariant=Disabled  NVariant=Disabled  NCopyVariant=Disabled_SignalSpec  FilterICVariant=Disabled  IntegratorICVariant=InternalICs  ExternalResetVariant=Disabled  TRSumVariant=Passthrough  SumFdbkVariant=Disabled  SumVariant=Sum_PI  TsampFilterVariant=InternalTs  TsampNgainVariant=Passthrough  TsampIntegralVariant=Disabled_SignalSpec  ExternalSaturationOutDataTypeStr=Inherit: Same as second input  DerivativeSourceVariant=Disabled  PreIntVariant=InternalPreInt
  nozzle angle : Outport
  wires:
  pitch/1 -> Add/1
  pitch_setpoint/1 -> Add/2
  Add/1 -> Pitch Controller/1
  Add1/1 -> Pitch Rate Controller/1
  pitch rate/1 -> Add1/1
  Pitch Controller/1 -> Add1/2
  Pitch Rate Controller/1 -> nozzle angle/1
